simulink model "sim_dist_att_obs_paper"  (R2020a)
settings: Solver=ode4  StartTime=0.0  StopTime=30.0  FixedStep=0.01  RelTol=1e-3
values from neighbouring files (symbols this model uses):
  beta_Phi_1 = pp0 * cal_frac_squ( 3, p_p0_plus_1, q_p0_plus_1 )                          * cal_frac_squ( eps_s_bar / pi, p_p0_min_2, q_p0_min_2 )                          / ( 2 * ( 2 * pp0 - 1 ) * tanh( gamma0 * ( eps_s_bar / pi ) / 2 ) )                          - ( cal_frac_squ( 3, p_p0_plus_1, q_p0_plus_1 ) * gamma0 / ( 4 * ( 2 * pp0 -1 ) ) )                          * cal_frac_squ( eps_s_bar / pi, p_p0_min_ ...(+136 chars)    [draw_compare_dist_att_obs.m]
  beta_Phi_2 = ( 1 - pp0 ) * cal_frac_squ( 3, p_p0_plus_1, q_p0_plus_1 )                          / ( 2 * ( 1 - 2 * pp0 ) * cal_frac_squ( eps_s_bar / pi, p_p0_0, q_p0_0 ) * tanh( gamma0 * ( eps_s_bar / pi ) / 2 ) )                          - ( cal_frac_squ( 3, p_p0_plus_1, q_p0_plus_1 ) * gamma0 / ( 4 * ( 1 - 2 * pp0 ) ) )                          * cal_frac_squ( eps_s_bar / pi, p_1_min_p0, q_1_min_p0 )          ...(+112 chars)    [draw_compare_dist_att_obs.m]
  c1_diff_sigma_bar_w = diag([12; 12; 12])    [draw_compare_dist_att_obs.m]
  c1_diff_ui = diag([25; 30; 20])    [draw_compare_dist_att_obs.m]
  c2_diff_sigma_bar_w = diag([12; 12; 12])    [draw_compare_dist_att_obs.m]
  c2_diff_ui = diag([50; 50; 10])    [draw_compare_dist_att_obs.m]
  c3_diff_sigma_bar_w = diag([15; 15; 15])    [draw_compare_dist_att_obs.m]
  c3_diff_ui = diag([15; 15; 10])    [draw_compare_dist_att_obs.m]
  c_w_1 = diag( [20; 15; 15] )    [draw_compare_dist_att_obs.m]
  c_w_2 = diag( [20; 15; 15] )    [draw_compare_dist_att_obs.m]
  c_w_3 = diag( [2; 2; 2] )    [draw_compare_dist_att_obs.m]
  cS0 = diag( [4.5; 4.5; 4.5] )    [draw_compare_dist_att_obs.m]
  dw_aa_t = 0.2 * ones(3, 5) + ( 1.0 - 0.2 ) * rand(3, 5)    [draw_compare_dist_att_obs.m]
  dw_ff_t = [ 0.4 * ones(1, 5) + ( 1.0 - 0.4 ) * rand(1, 5);                      0.4 * ones(1, 5) + ( 1.0 - 0.4 ) * rand(1, 5);                      0.2 * ones(1, 5) + ( 0.6 - 0.2 ) * rand(1, 5) ]    [draw_compare_dist_att_obs.m]
  dw_phi_t = ( - pi / 2 ) * ones(3, 5) + ( pi / 2 - ( - pi / 2 ) ) * rand(3, 5)    [draw_compare_dist_att_obs.m]
  dwci_init = zeros(3,5)    [draw_compare_dist_att_obs.m]
  eps_s_bar_div_pi = eps_s_bar / pi    (= 0.03)    [draw_compare_dist_att_obs.m]
  gamma0 = 20    [draw_compare_dist_att_obs.m]
  h1w = diag([20.0; 20.0; 20.0])    [draw_compare_dist_att_obs.m]
  h2w = diag([30.0; 35.0; 35.0])    [draw_compare_dist_att_obs.m]
  h3w = diag([30.0; 25.0; 30.0])    [draw_compare_dist_att_obs.m]
  Ji = zeros(3,3,NF)    [draw_compare_dist_att_obs.m]
  k_J_0 = diag( [1; 1; 1] )    [draw_compare_dist_att_obs.m]
  Lamd_diff_sigma_bar_w = 0.8    [draw_compare_dist_att_obs.m]
  Lamd_diff_ui = 0.8    [draw_compare_dist_att_obs.m]
  mu_c_theta = 100    [draw_compare_dist_att_obs.m]
  mu_d_w = 100    [draw_compare_dist_att_obs.m]
  pos0 = zeros(3, 1)    [draw_compare_dist_att_obs.m]
  pp0 = 8 / 11    (= 0.727272727273)    [draw_compare_dist_att_obs.m]
  PZ0 = P0(3)    [draw_compare_dist_att_obs.m]
  PZ1 = 10    [draw_compare_dist_att_obs.m]
  Qci_init = repmat([1;0;0;0],1,NF)    [draw_compare_dist_att_obs.m]
  R0 = 4    [draw_compare_dist_att_obs.m]
  R1 = 8    [draw_compare_dist_att_obs.m]
  Rci_init = zeros(3,3,NF)    [draw_compare_dist_att_obs.m]
  Ri_init = zeros(3,3,NF)    [draw_compare_dist_att_obs.m]
  Rx2 = 10    [draw_compare_dist_att_obs.m]
  Ry2 = 6    [draw_compare_dist_att_obs.m]
  Rz2 = 4    [draw_compare_dist_att_obs.m]
  T0 = 0    [draw_compare_dist_att_obs.m]
  T1 = tseq1    (= 10)    [draw_compare_dist_att_obs.m]
  T2 = tseq1 + tseq12 + tseq2    (= 30)    [draw_compare_dist_att_obs.m]
  thr_p_plus_1 = cal_frac_squ( 3, p_p0_plus_1, q_p0_plus_1 )    [draw_compare_dist_att_obs.m]
  ui_init = zeros(3,NF)    [draw_compare_dist_att_obs.m]
  vel0 = zeros(3, 1)    [draw_compare_dist_att_obs.m]
  wci_init = zeros(3,5)    [draw_compare_dist_att_obs.m]
  zeta_diff_sigma_bar_w = 0.3    [draw_compare_dist_att_obs.m]
  zeta_diff_ui = 0.05    [draw_compare_dist_att_obs.m]
undefined symbols (not defined in the file or in its folder): cal_frac_squ, p_2_p0, p_alfaw1, p_alfaw2, p_beta_w_1, p_beta_w_2, p_p0_min_1, p_p0_plus_1, q_2_p0, q_alfaw1, q_alfaw2, q_beta_w_1, q_beta_w_2, q_p0_min_1, q_p0_plus_1, Qei_init, Qi_init, Rei_init, V_Phi_Rei_init, wei_init, wi_init
(part 1 of 5)
settings Model: Creator=zzy  LastModifiedBy=Hershey.A
settings DataIOCC: ReturnWorkspaceOutputs=off
settings DebuggingCC: ArithmeticOperatorsInVariantConditions=warning
settings SFSimCC: SimUseLocalCustomCode=off  CustomCodeUndefinedFunction=UseInterfaceOnly
settings RTWCC: RTWUseLocalCustomCode=off

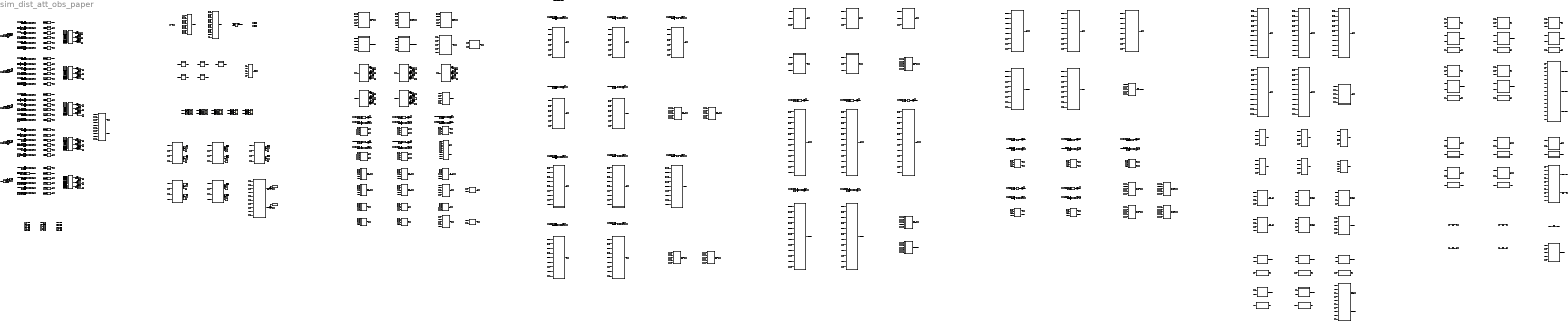
== system sim_dist_att_obs_paper ==
  Abs{,1..29} (30 alike) : Abs
  Add{10..12,14,16..18,20..22,24..26,28..29} (15 alike) : Sum
  Add{13,15,19,23,27} (5 alike) : Sum  Inputs=+-
  Clock : Clock
  Constant : Constant  Value=T1
  Constant129 : Constant  Value=R0
  Constant130 : Constant  Value=R1
  Constant131 : Constant  Value=T0
  Constant132 : Constant  Value=Rz2
  Constant133 : Constant  Value=Ry2
  Constant134 : Constant  Value=Rx2
  Constant{298,331,362,619,639} (5 alike) : Constant  Value=0
  Constant{299,411,488,556,621} (5 alike) : Constant  Value=p_p0_plus_1
  Constant{300,355,433,510,521} (5 alike) : Constant  Value=p_2_p0
  Constant{301,306,308,310,316,321,324,326,343,347,352,354,357,363,590,593,598,601,603,620,624,629,631,634,640} (25 alike) : Constant
  Constant{302,309,312..313,317,325,327..328,345..346,348,356,358..359,364..365,591..592,594,602,615..616,622..623,625,633,635..636,641..642} (30 alike) : Constant  Value=3
  Constant{303,314,318,329,349,360,595,617,626,637} (10 alike) : Constant  Value=2
  Constant{304,319,350,596,627} (5 alike) : Constant  Value=c1_diff_ui
  Constant{305,320,351,597,628} (5 alike) : Constant  Value=c2_diff_ui
  Constant{307,323,353,600,630} (5 alike) : Constant  Value=c3_diff_ui
  Constant{311,366,444,522,577} (5 alike) : Constant  Value=q_2_p0
  Constant{315,330,361,618,638} (5 alike) : Constant  Value=Lamd_diff_ui
  Constant{322,377,455,483,485,487,490,492,533,588,609,611..614} (15 alike) : Constant  Value=cS0
  Constant{332,335,337,339,341} (5 alike) : Constant  Value=p_p0_min_1
  Constant{333,388,393,461,466,468,474,481,544..545,578,583,589,599,607} (15 alike) : Constant  Value=gamma0
  Constant{334,336,338,340,342} (5 alike) : Constant  Value=q_p0_min_1
  Constant{344,392,398..399,467,473,477,480,547,555,575,581,586,605,610} (15 alike) : Constant  Value=thr_p_plus_1
  Constant{367..376,378..382} (15 alike) : Constant  Value=zeta_diff_ui
  Constant{383..387,401,413,437,447,450..452,454,457,459,484,486,489,491,493,526,530,535,539,543} (25 alike) : Constant  Value=Ji
  Constant{389,395,463,470,476} (5 alike) : Constant  Value=pp0
  Constant{390,396,464,471,478,571,579,584,604,608} (10 alike) : Constant  Value=beta_Phi_1
  Constant{391,397,465,472,479,548..549,574,580,585} (10 alike) : Constant  Value=beta_Phi_2
  Constant{394,462,469,475,482,546,576,582,587,606} (10 alike) : Constant  Value=eps_s_bar_div_pi
  Constant{400,425,445..446,448..449,453,456,458,460} (10 alike) : Constant  Value=h3w
  Constant{402,404,409,417,423} (5 alike) : Constant  Value=p_alfaw1
  Constant{403,405,412,418,424} (5 alike) : Constant  Value=mu_d_w
  Constant{406,414,419,426,429} (5 alike) : Constant  Value=q_alfaw1
  Constant{407,415,420,427,430} (5 alike) : Constant  Value=p_alfaw2
  Constant{408,416,421,428,431} (5 alike) : Constant  Value=q_alfaw2
  Constant{410,422,499,560,632} (5 alike) : Constant  Value=q_p0_plus_1
  Constant{432,435,438,440,442} (5 alike) : Constant  Value=h1w
  Constant{434,436,439,441,443} (5 alike) : Constant  Value=h2w
  Constant{494,500,505,511,516} (5 alike) : Constant  Value=p_beta_w_1
  Constant{495,501,506,512,517} (5 alike) : Constant  Value=q_beta_w_1
  Constant{496,502,507,513,518} (5 alike) : Constant  Value=p_beta_w_2
  Constant{497,503,508,514,519} (5 alike) : Constant  Value=q_beta_w_2
  Constant{498,504,509,515,520} (5 alike) : Constant  Value=mu_c_theta
  Constant{523,527,531,536,540} (5 alike) : Constant  Value=c_w_1
  Constant{524,528,532,537,541} (5 alike) : Constant  Value=c_w_2
  Constant{525,529,534,538,542} (5 alike) : Constant  Value=c_w_3
  Constant{550..554} (5 alike) : Constant  Value=k_J_0
  Constant{557,561,564,567,570} (5 alike) : Constant  Value=dw_aa_t
  Constant{558,562,565,568,572} (5 alike) : Constant  Value=dw_ff_t
  Constant{559,563,566,569,573} (5 alike) : Constant  Value=dw_phi_t
  Constant64 : Constant  Value=T2
  Constant65 : Constant  Value=R0
  Constant66 : Constant  Value=R1
  Constant67 : Constant  Value=Rx2
  Constant68 : Constant  Value=Ry2
  Constant69 : Constant  Value=Rz2
  Constant70 : Constant  Value=T2
  Constant71 : Constant  Value=T1
  Constant72 : Constant  Value=PZ0
  Constant73 : Constant  Value=PZ1
  Demux{,1,22,98..141} (47 alike) : Demux  Outputs=3
  Display{96..172} (77 alike) : Display
  Integrator{1..15,46..50} (20 alike) : Integrator  InitialCondition=zeros(3,1)
  Integrator17 : Integrator  InitialCondition=V_Phi_Rei_init(:,2)
  Integrator19 : Integrator  InitialCondition=V_Phi_Rei_init(:,3)
  Integrator20 : Integrator  InitialCondition=V_Phi_Rei_init(:,1)
  Integrator21 : Integrator  InitialCondition=wi_init(:,1)
  Integrator22 : Integrator  InitialCondition=wi_init(:,2)
  Integrator23 : Integrator  InitialCondition=wi_init(:,3)
  Integrator24 : Integrator  InitialCondition=wi_init(:,4)
  Integrator25 : Integrator  InitialCondition=wi_init(:,5)
  Integrator26 : Integrator  InitialCondition=Qi_init(:,1)
  Integrator27 : Integrator  InitialCondition=Qi_init(:,2)
  Integrator28 : Integrator  InitialCondition=Qi_init(:,3)
  Integrator29 : Integrator  InitialCondition=Qi_init(:,4)
  Integrator30 : Integrator  InitialCondition=Qi_init(:,5)
  Integrator31 : Integrator  InitialCondition=Qei_init(:,1)
  Integrator32 : Integrator  InitialCondition=Qei_init(:,2)
  Integrator33 : Integrator  InitialCondition=Qei_init(:,3)
  Integrator34 : Integrator  InitialCondition=Qei_init(:,4)
  Integrator35 : Integrator  InitialCondition=Qei_init(:,5)
  Integrator42 : Integrator  InitialCondition=V_Phi_Rei_init(:,4)
  Integrator44 : Integrator  InitialCondition=V_Phi_Rei_init(:,5)
  Interpreted MATLAB Function{,61..124} (65 alike) : MATLABFcn  MATLABFcn=cal_frac_squ(u(1:3),u(4),u(5))
  Memory : Memory  InitialCondition=ui_init
  Memory{9..11,13,18..25} (12 alike) : Memory  InitialCondition=zeros(3,5)
  Memory12 : Memory  InitialCondition=V_Phi_Rei_init
  Memory14 : Memory  InitialCondition=wci_init
  Memory15 : Memory  InitialCondition=dwci_init
  Memory16 : Memory  InitialCondition=Qci_init
  Memory17 : Memory  InitialCondition=Rci_init
  Memory3 : Memory  InitialCondition=Qi_init
  Memory4 : Memory  InitialCondition=Ri_init
  Memory5 : Memory  InitialCondition=wi_init
  Memory6 : Memory  InitialCondition=wei_init
  Memory7 : Memory  InitialCondition=Qei_init
  Memory8 : Memory  InitialCondition=Rei_init
  Mux{136..170,180,187..215} (65 alike) : Mux  Inputs=3
  Mux{171..179,181..186} (15 alike) : Mux  Inputs=2
  Product{,1..9} (10 alike) : Product
  Qei dynam agent 1 : MATLAB Function  TreatAsAtomicUnit=on
  Qei dynam agent 2 : MATLAB Function  TreatAsAtomicUnit=on
  Qei dynam agent 3 : MATLAB Function  TreatAsAtomicUnit=on
  Qei dynam agent 4 : MATLAB Function  TreatAsAtomicUnit=on
  Qei dynam agent 5 : MATLAB Function  TreatAsAtomicUnit=on
  Qi dynam agent 1 : MATLAB Function  TreatAsAtomicUnit=on
  Qi dynam agent 2 : MATLAB Function  TreatAsAtomicUnit=on
  Qi dynam agent 3 : MATLAB Function  TreatAsAtomicUnit=on
  Qi dynam agent 4 : MATLAB Function  TreatAsAtomicUnit=on
  Qi dynam agent 5 : MATLAB Function  TreatAsAtomicUnit=on
  Scope{1..2,13..15} (5 alike) : Scope  NumInputPorts=3
  Step : Step  Time=T1+0.01  SampleTime=0
  To Workspace23 : ToWorkspace  VariableName=wci  SampleTime=-1
  To Workspace24 : ToWorkspace  VariableName=V_Phi_Rei  SampleTime=-1
  To Workspace25 : ToWorkspace  VariableName=dwi_tilt  SampleTime=-1
  To Workspace26 : ToWorkspace  VariableName=Qci  SampleTime=-1
  To Workspace27 : ToWorkspace  VariableName=sigma_bar_w_hat  SampleTime=-1
  To Workspace28 : ToWorkspace  VariableName=wei  SampleTime=-1
  To Workspace29 : ToWorkspace  VariableName=sigma_w  SampleTime=-1
  To Workspace30 : ToWorkspace  VariableName=sigma_bar_w  SampleTime=-1
  To Workspace31 : ToWorkspace  VariableName=Phi_psi_e  SampleTime=-1
  To Workspace32 : ToWorkspace  VariableName=Phi_bar_psi_e  SampleTime=-1
  To Workspace33 : ToWorkspace  VariableName=Qei  SampleTime=-1
  To Workspace34 : ToWorkspace  VariableName=wi  SampleTime=-1
  To Workspace35 : ToWorkspace  VariableName=Qi  SampleTime=-1
  To Workspace36 : ToWorkspace  VariableName=S_bar  SampleTime=-1
  To Workspace37 : ToWorkspace  VariableName=Si  SampleTime=-1
  To Workspace38 : ToWorkspace  VariableName=dwi  SampleTime=-1
  To Workspace39 : ToWorkspace  VariableName=dwi_hat  SampleTime=-1
  cal Fi_S agent 1 : MATLAB Function  TreatAsAtomicUnit=on
  cal Fi_S agent 2 : MATLAB Function  TreatAsAtomicUnit=on
  cal Fi_S agent 3 : MATLAB Function  TreatAsAtomicUnit=on
  cal Fi_S agent 4 : MATLAB Function  TreatAsAtomicUnit=on
  cal Fi_S agent 5 : MATLAB Function  TreatAsAtomicUnit=on
  cal Phi_bar_psi_e agent 1 : MATLAB Function  TreatAsAtomicUnit=on
  cal Phi_bar_psi_e agent 2 : MATLAB Function  TreatAsAtomicUnit=on
  cal Phi_bar_psi_e agent 3 : MATLAB Function  TreatAsAtomicUnit=on
  cal Phi_bar_psi_e agent 4 : MATLAB Function  TreatAsAtomicUnit=on
  cal Phi_bar_psi_e agent 5 : MATLAB Function  TreatAsAtomicUnit=on
  cal Phi_psi_e agent 1 : MATLAB Function  TreatAsAtomicUnit=on
  cal Phi_psi_e agent 2 : MATLAB Function  TreatAsAtomicUnit=on
  cal Phi_psi_e agent 3 : MATLAB Function  TreatAsAtomicUnit=on
  cal Phi_psi_e agent 4 : MATLAB Function  TreatAsAtomicUnit=on
  cal Phi_psi_e agent 5 : MATLAB Function  TreatAsAtomicUnit=on
  cal Qci agent 1 : MATLAB Function  TreatAsAtomicUnit=on
  cal Qci agent 2 : MATLAB Function  TreatAsAtomicUnit=on
  cal Qci agent 3 : MATLAB Function  TreatAsAtomicUnit=on
  cal Qci agent 4 : MATLAB Function  TreatAsAtomicUnit=on
  cal Qci agent 5 : MATLAB Function  TreatAsAtomicUnit=on
  cal Rci agent 1 : MATLAB Function  TreatAsAtomicUnit=on
  cal Rci agent 2 : MATLAB Function  TreatAsAtomicUnit=on
  cal Rci agent 3 : MATLAB Function  TreatAsAtomicUnit=on
  cal Rci agent 4 : MATLAB Function  TreatAsAtomicUnit=on
  cal Rci agent 5 : MATLAB Function  TreatAsAtomicUnit=on
  cal Rei agent 1 : MATLAB Function  TreatAsAtomicUnit=on
  cal Rei agent 2 : MATLAB Function  TreatAsAtomicUnit=on
  cal Rei agent 3 : MATLAB Function  TreatAsAtomicUnit=on
  cal Rei agent 4 : MATLAB Function  TreatAsAtomicUnit=on
  cal Rei agent 5 : MATLAB Function  TreatAsAtomicUnit=on
  cal Ri agent 1 : MATLAB Function  TreatAsAtomicUnit=on
  cal Ri agent 2 : MATLAB Function  TreatAsAtomicUnit=on
  cal Ri agent 3 : MATLAB Function  TreatAsAtomicUnit=on
  cal Ri agent 4 : MATLAB Function  TreatAsAtomicUnit=on
  cal Ri agent 5 : MATLAB Function  TreatAsAtomicUnit=on
  cal S_bar agent 1 : MATLAB Function  TreatAsAtomicUnit=on
  cal S_bar agent 2 : MATLAB Function  TreatAsAtomicUnit=on
  cal S_bar agent 3 : MATLAB Function  TreatAsAtomicUnit=on
  cal S_bar agent 4 : MATLAB Function  TreatAsAtomicUnit=on
  cal S_bar agent 5 : MATLAB Function  TreatAsAtomicUnit=on
  cal Si agent 1 : MATLAB Function  TreatAsAtomicUnit=on
  cal Si agent 2 : MATLAB Function  TreatAsAtomicUnit=on
  cal Si agent 3 : MATLAB Function  TreatAsAtomicUnit=on
  cal Si agent 4 : MATLAB Function  TreatAsAtomicUnit=on
  cal Si agent 5 : MATLAB Function  TreatAsAtomicUnit=on
  cal abs 61 : MATLAB Function  TreatAsAtomicUnit=on
  cal abs 62 : MATLAB Function  TreatAsAtomicUnit=on
  cal abs 63 : MATLAB Function  TreatAsAtomicUnit=on
  cal abs 64 : MATLAB Function  TreatAsAtomicUnit=on
  cal abs 65 : MATLAB Function  TreatAsAtomicUnit=on
  cal abs 66 : MATLAB Function  TreatAsAtomicUnit=on
  cal abs 67 : MATLAB Function  TreatAsAtomicUnit=on
  cal abs 68 : MATLAB Function  TreatAsAtomicUnit=on
  cal abs 69 : MATLAB Function  TreatAsAtomicUnit=on
  cal abs 70 : MATLAB Function  TreatAsAtomicUnit=on
  cal abs 71 : MATLAB Function  TreatAsAtomicUnit=on
  cal abs 72 : MATLAB Function  TreatAsAtomicUnit=on
  cal abs 73 : MATLAB Function  TreatAsAtomicUnit=on
  cal abs 74 : MATLAB Function  TreatAsAtomicUnit=on
  cal abs 75 : MATLAB Function  TreatAsAtomicUnit=on
  cal abs 76 : MATLAB Function  TreatAsAtomicUnit=on
  cal abs 77 : MATLAB Function  TreatAsAtomicUnit=on
  cal abs 78 : MATLAB Function  TreatAsAtomicUnit=on
  cal abs 79 : MATLAB Function  TreatAsAtomicUnit=on
  cal abs 80 : MATLAB Function  TreatAsAtomicUnit=on
  cal abs 81 : MATLAB Function  TreatAsAtomicUnit=on
  cal abs 82 : MATLAB Function  TreatAsAtomicUnit=on
  cal abs 83 : MATLAB Function  TreatAsAtomicUnit=on
  cal abs 84 : MATLAB Function  TreatAsAtomicUnit=on
  cal abs 85 : MATLAB Function  TreatAsAtomicUnit=on
  cal abs 86 : MATLAB Function  TreatAsAtomicUnit=on
  cal abs 87 : MATLAB Function  TreatAsAtomicUnit=on
  cal abs 88 : MATLAB Function  TreatAsAtomicUnit=on
  cal abs 89 : MATLAB Function  TreatAsAtomicUnit=on
  cal abs 90 : MATLAB Function  TreatAsAtomicUnit=on
  cal abs 91 : MATLAB Function  TreatAsAtomicUnit=on
  cal abs 92 : MATLAB Function  TreatAsAtomicUnit=on
  cal abs 93 : MATLAB Function  TreatAsAtomicUnit=on
  cal abs 94 : MATLAB Function  TreatAsAtomicUnit=on
  cal abs 95 : MATLAB Function  TreatAsAtomicUnit=on
  cal combine sigma_bar_w_tilt : MATLAB Function  TreatAsAtomicUnit=on
  cal d_sigma_w agent 1 : MATLAB Function  TreatAsAtomicUnit=on
  cal d_sigma_w agent 2 : MATLAB Function  TreatAsAtomicUnit=on
  cal d_sigma_w agent 3 : MATLAB Function  TreatAsAtomicUnit=on
  cal d_sigma_w agent 4 : MATLAB Function  TreatAsAtomicUnit=on
  cal d_sigma_w agent 5 : MATLAB Function  TreatAsAtomicUnit=on
  cal d_theta_hat : MATLAB Function  TreatAsAtomicUnit=on
  cal d_theta_hat1 : MATLAB Function  TreatAsAtomicUnit=on
  cal d_theta_hat2 : MATLAB Function  TreatAsAtomicUnit=on
  cal d_theta_hat3 : MATLAB Function  TreatAsAtomicUnit=on
  cal d_theta_hat4 : MATLAB Function  TreatAsAtomicUnit=on
  cal differentiator d_sigma_bar_w_hat agent 1 : Subsystem
  cal differentiator d_sigma_bar_w_hat agent 2 : Subsystem
  cal differentiator d_sigma_bar_w_hat agent 3 : Subsystem
  cal differentiator d_sigma_bar_w_hat agent 4 : Subsystem
  cal differentiator d_sigma_bar_w_hat agent 5 : Subsystem
  cal divide pi : MATLAB Function  TreatAsAtomicUnit=on
  cal dw_hat agent 1 : MATLAB Function  TreatAsAtomicUnit=on
  cal dw_hat agent 2 : MATLAB Function  TreatAsAtomicUnit=on
  cal dw_hat agent 3 : MATLAB Function  TreatAsAtomicUnit=on
  cal dw_hat agent 4 : MATLAB Function  TreatAsAtomicUnit=on
  cal dw_hat agent 5 : MATLAB Function  TreatAsAtomicUnit=on
  cal error dw_tilt : MATLAB Function  TreatAsAtomicUnit=on
  cal sig : MATLAB Function  TreatAsAtomicUnit=on
  cal sig1 : MATLAB Function  TreatAsAtomicUnit=on
  cal sig10 : MATLAB Function  TreatAsAtomicUnit=on
  cal sig11 : MATLAB Function  TreatAsAtomicUnit=on
  cal sig12 : MATLAB Function  TreatAsAtomicUnit=on
  cal sig13 : MATLAB Function  TreatAsAtomicUnit=on
  cal sig14 : MATLAB Function  TreatAsAtomicUnit=on
  cal sig15 : MATLAB Function  TreatAsAtomicUnit=on
  cal sig16 : MATLAB Function  TreatAsAtomicUnit=on
  cal sig17 : MATLAB Function  TreatAsAtomicUnit=on
  cal sig18 : MATLAB Function  TreatAsAtomicUnit=on
  cal sig19 : MATLAB Function  TreatAsAtomicUnit=on
  cal sig2 : MATLAB Function  TreatAsAtomicUnit=on
  cal sig20 : MATLAB Function  TreatAsAtomicUnit=on
  cal sig21 : MATLAB Function  TreatAsAtomicUnit=on
  cal sig22 : MATLAB Function  TreatAsAtomicUnit=on
  cal sig23 : MATLAB Function  TreatAsAtomicUnit=on
  cal sig24 : MATLAB Function  TreatAsAtomicUnit=on
  cal sig25 : MATLAB Function  TreatAsAtomicUnit=on
  cal sig26 : MATLAB Function  TreatAsAtomicUnit=on
  cal sig27 : MATLAB Function  TreatAsAtomicUnit=on
  cal sig28 : MATLAB Function  TreatAsAtomicUnit=on
  cal sig29 : MATLAB Function  TreatAsAtomicUnit=on
  cal sig3 : MATLAB Function  TreatAsAtomicUnit=on
  cal sig4 : MATLAB Function  TreatAsAtomicUnit=on
  cal sig5 : MATLAB Function  TreatAsAtomicUnit=on
  cal sig6 : MATLAB Function  TreatAsAtomicUnit=on
  cal sig7 : MATLAB Function  TreatAsAtomicUnit=on
  cal sig8 : MATLAB Function  TreatAsAtomicUnit=on
  cal sig9 : MATLAB Function  TreatAsAtomicUnit=on
  cal sigma_bar_w_hat agent 1 : MATLAB Function  TreatAsAtomicUnit=on
  cal sigma_bar_w_hat agent 2 : MATLAB Function  TreatAsAtomicUnit=on
  cal sigma_bar_w_hat agent 3 : MATLAB Function  TreatAsAtomicUnit=on
  cal sigma_bar_w_hat agent 4 : MATLAB Function  TreatAsAtomicUnit=on
  cal sigma_bar_w_hat agent 5 : MATLAB Function  TreatAsAtomicUnit=on
  cal sigma_w_bar : MATLAB Function  TreatAsAtomicUnit=on
  cal taui agent 1 : MATLAB Function  TreatAsAtomicUnit=on
  cal taui agent 2 : MATLAB Function  TreatAsAtomicUnit=on
  cal taui agent 3 : MATLAB Function  TreatAsAtomicUnit=on
  cal taui agent 4 : MATLAB Function  TreatAsAtomicUnit=on
  cal taui agent 5 : MATLAB Function  TreatAsAtomicUnit=on
  cal theta_Si_beta_w agent 1 : MATLAB Function  TreatAsAtomicUnit=on
  cal theta_Si_beta_w agent 2 : MATLAB Function  TreatAsAtomicUnit=on
  cal theta_Si_beta_w agent 3 : MATLAB Function  TreatAsAtomicUnit=on
  cal theta_Si_beta_w agent 4 : MATLAB Function  TreatAsAtomicUnit=on
  cal theta_Si_beta_w agent 5 : MATLAB Function  TreatAsAtomicUnit=on
  cal theta_sigma_bar_w_tilt agent 1 : MATLAB Function  TreatAsAtomicUnit=on
  cal theta_sigma_bar_w_tilt agent 2 : MATLAB Function  TreatAsAtomicUnit=on
  cal theta_sigma_bar_w_tilt agent 3 : MATLAB Function  TreatAsAtomicUnit=on
  cal theta_sigma_bar_w_tilt agent 4 : MATLAB Function  TreatAsAtomicUnit=on
  cal theta_sigma_bar_w_tilt agent 5 : MATLAB Function  TreatAsAtomicUnit=on
  cal wci dwci agent 1 : MATLAB Function  TreatAsAtomicUnit=on
  cal wci dwci agent 2 : MATLAB Function  TreatAsAtomicUnit=on
  cal wci dwci agent 3 : MATLAB Function  TreatAsAtomicUnit=on
  cal wci dwci agent 4 : MATLAB Function  TreatAsAtomicUnit=on
  cal wci dwci agent 5 : MATLAB Function  TreatAsAtomicUnit=on
  cal wei agent 1 : MATLAB Function  TreatAsAtomicUnit=on
  cal wei agent 2 : MATLAB Function  TreatAsAtomicUnit=on
  cal wei agent 3 : MATLAB Function  TreatAsAtomicUnit=on
  cal wei agent 4 : MATLAB Function  TreatAsAtomicUnit=on
  cal wei agent 5 : MATLAB Function  TreatAsAtomicUnit=on
  choose ksi_est_err 41 : MATLAB Function  TreatAsAtomicUnit=on
  choose ksi_est_err 42 : MATLAB Function  TreatAsAtomicUnit=on
  choose ksi_est_err 43 : MATLAB Function  TreatAsAtomicUnit=on
  choose ksi_est_err 44 : MATLAB Function  TreatAsAtomicUnit=on
  choose ksi_est_err 45 : MATLAB Function  TreatAsAtomicUnit=on
  choose ksi_est_err 46 : MATLAB Function  TreatAsAtomicUnit=on
  choose ksi_est_err 47 : MATLAB Function  TreatAsAtomicUnit=on
  choose ksi_est_err 48 : MATLAB Function  TreatAsAtomicUnit=on
  choose ksi_est_err 49 : MATLAB Function  TreatAsAtomicUnit=on
  choose ksi_est_err 50 : MATLAB Function  TreatAsAtomicUnit=on
  choose ksi_est_err 51 : MATLAB Function  TreatAsAtomicUnit=on
  choose ksi_est_err 52 : MATLAB Function  TreatAsAtomicUnit=on
  choose ksi_est_err 53 : MATLAB Function  TreatAsAtomicUnit=on
  choose ksi_est_err 54 : MATLAB Function  TreatAsAtomicUnit=on
  choose ksi_est_err 55 : MATLAB Function  TreatAsAtomicUnit=on
  choose ksi_est_err 56 : MATLAB Function  TreatAsAtomicUnit=on
  choose ksi_est_err 57 : MATLAB Function  TreatAsAtomicUnit=on
  choose ksi_est_err 58 : MATLAB Function  TreatAsAtomicUnit=on
  choose ksi_est_err 59 : MATLAB Function  TreatAsAtomicUnit=on
  choose ksi_est_err 60 : MATLAB Function  TreatAsAtomicUnit=on
  choose ksi_est_err 61 : MATLAB Function  TreatAsAtomicUnit=on
  choose ksi_est_err 62 : MATLAB Function  TreatAsAtomicUnit=on
  choose ksi_est_err 63 : MATLAB Function  TreatAsAtomicUnit=on
  choose ksi_est_err 64 : MATLAB Function  TreatAsAtomicUnit=on
  choose ksi_est_err 65 : MATLAB Function  TreatAsAtomicUnit=on
  choose ksi_est_err 66 : MATLAB Function  TreatAsAtomicUnit=on
  choose ksi_est_err 67 : MATLAB Function  TreatAsAtomicUnit=on
  choose ksi_est_err 68 : MATLAB Function  TreatAsAtomicUnit=on
  choose ksi_est_err 69 : MATLAB Function  TreatAsAtomicUnit=on
  choose ksi_est_err 70 : MATLAB Function  TreatAsAtomicUnit=on
  choose ksi_est_err 71 : MATLAB Function  TreatAsAtomicUnit=on
  choose ksi_est_err 72 : MATLAB Function  TreatAsAtomicUnit=on
  choose ksi_est_err 73 : MATLAB Function  TreatAsAtomicUnit=on
  choose ksi_est_err 74 : MATLAB Function  TreatAsAtomicUnit=on
  choose ksi_est_err 75 : MATLAB Function  TreatAsAtomicUnit=on
  choose ui agent 1 : MATLAB Function  TreatAsAtomicUnit=on
  choose ui agent 2 : MATLAB Function  TreatAsAtomicUnit=on
  choose ui agent 3 : MATLAB Function  TreatAsAtomicUnit=on
  choose ui agent 4 : MATLAB Function  TreatAsAtomicUnit=on
  choose ui agent 5 : MATLAB Function  TreatAsAtomicUnit=on
  combine Fi_S : MATLAB Function  TreatAsAtomicUnit=on
  combine Phi_bar_psi_e : MATLAB Function  TreatAsAtomicUnit=on
  combine Phi_psi_e : MATLAB Function  TreatAsAtomicUnit=on
  combine Qci Rci : MATLAB Function  TreatAsAtomicUnit=on
  combine Qci Rci1 : MATLAB Function  TreatAsAtomicUnit=on
  combine Qi Ri : MATLAB Function  TreatAsAtomicUnit=on
  combine S_bar : MATLAB Function  TreatAsAtomicUnit=on
  combine Si : MATLAB Function  TreatAsAtomicUnit=on
  combine Si_squ_beta_w_1 : MATLAB Function  TreatAsAtomicUnit=on
  combine Si_squ_beta_w_2 : MATLAB Function  TreatAsAtomicUnit=on
  combine V_Phi_Rei_squ_2p : MATLAB Function  TreatAsAtomicUnit=on
  combine V_Phi_Rei_squ_p_min_1 : MATLAB Function  TreatAsAtomicUnit=on
  combine V_Phi_Rei_squ_p_plus_1 : MATLAB Function  TreatAsAtomicUnit=on
  combine d_sigma_bar_v_est1 : MATLAB Function  TreatAsAtomicUnit=on
  combine duihat d2uihat : MATLAB Function  TreatAsAtomicUnit=on
  combine dw_hat : MATLAB Function  TreatAsAtomicUnit=on
  combine dwi : MATLAB Function  TreatAsAtomicUnit=on
  combine norminal formation control input : MATLAB Function  TreatAsAtomicUnit=on
  combine sigma_bar_w_hat : MATLAB Function  TreatAsAtomicUnit=on
  combine sigma_w : MATLAB Function  TreatAsAtomicUnit=on
  combine tau : MATLAB Function  TreatAsAtomicUnit=on
  combine tau1 : MATLAB Function  TreatAsAtomicUnit=on
  combine theta_Si_beta_w_1 : MATLAB Function  TreatAsAtomicUnit=on
  combine theta_Si_beta_w_2 : MATLAB Function  TreatAsAtomicUnit=on
  combine theta_sigma_bar_w_tilt : MATLAB Function  TreatAsAtomicUnit=on
  combine wci dwci : MATLAB Function  TreatAsAtomicUnit=on
  combine wei Qei Rei : MATLAB Function  TreatAsAtomicUnit=on
  control input generator agent 1 : MATLAB Function  TreatAsAtomicUnit=on
  control input generator agent 2 : MATLAB Function  TreatAsAtomicUnit=on
  control input generator agent 3 : MATLAB Function  TreatAsAtomicUnit=on
  control input generator agent 4 : MATLAB Function  TreatAsAtomicUnit=on
  control input generator agent 5 : MATLAB Function  TreatAsAtomicUnit=on
  d2_sigma_bar_w_est_{1..5} (5 alike) : Scope  NumInputPorts=3
  d2_ui_hat_node_{1..5} (5 alike) : Scope  NumInputPorts=3
  d_sigma_bar_w_est_{1..5} (5 alike) : Scope  NumInputPorts=3
  d_ui_hat_node_{1..5} (5 alike) : Scope  NumInputPorts=3
  dwci_node_{1..5} (5 alike) : Scope  NumInputPorts=3
  eta_0 : Scope  NumInputPorts=3
  generate angular rate disturbance agent 1 : MATLAB Function  TreatAsAtomicUnit=on
  generate angular rate disturbance agent 2 : MATLAB Function  TreatAsAtomicUnit=on
  generate angular rate disturbance agent 3 : MATLAB Function  TreatAsAtomicUnit=on
  generate angular rate disturbance agent 4 : MATLAB Function  TreatAsAtomicUnit=on
  generate angular rate disturbance agent 5 : MATLAB Function  TreatAsAtomicUnit=on
  ksi_0 : Scope  NumInputPorts=3
  leader control input : MATLAB Function  TreatAsAtomicUnit=on
  leader eta0 Integrator : Integrator  ExternalReset=rising  InitialConditionSource=external  InitialCondition=vel0
  leader ksi0 Integrator : Integrator  InitialCondition=pos0
  process velocity : MATLAB Function  TreatAsAtomicUnit=on
  sigma_bar_w_hat Integrator {1..5} (5 alike) : Integrator  InitialCondition=zeros(3,1)
  trans to column100 : MATLAB Function  TreatAsAtomicUnit=on
  trans to column101 : MATLAB Function  TreatAsAtomicUnit=on
  trans to column102 : MATLAB Function  TreatAsAtomicUnit=on
  trans to column103 : MATLAB Function  TreatAsAtomicUnit=on
  trans to column104 : MATLAB Function  TreatAsAtomicUnit=on
  trans to column105 : MATLAB Function  TreatAsAtomicUnit=on
  trans to column106 : MATLAB Function  TreatAsAtomicUnit=on
  trans to column107 : MATLAB Function  TreatAsAtomicUnit=on
  trans to column108 : MATLAB Function  TreatAsAtomicUnit=on
  trans to column109 : MATLAB Function  TreatAsAtomicUnit=on
  trans to column110 : MATLAB Function  TreatAsAtomicUnit=on
  trans to column111 : MATLAB Function  TreatAsAtomicUnit=on
  trans to column112 : MATLAB Function  TreatAsAtomicUnit=on
  trans to column113 : MATLAB Function  TreatAsAtomicUnit=on
  trans to column114 : MATLAB Function  TreatAsAtomicUnit=on
  trans to column115 : MATLAB Function  TreatAsAtomicUnit=on
  trans to column116 : MATLAB Function  TreatAsAtomicUnit=on
  trans to column117 : MATLAB Function  TreatAsAtomicUnit=on
  trans to column118 : MATLAB Function  TreatAsAtomicUnit=on
  trans to column119 : MATLAB Function  TreatAsAtomicUnit=on
  trans to column120 : MATLAB Function  TreatAsAtomicUnit=on
  trans to column121 : MATLAB Function  TreatAsAtomicUnit=on
  trans to column122 : MATLAB Function  TreatAsAtomicUnit=on
  trans to column123 : MATLAB Function  TreatAsAtomicUnit=on
  trans to column124 : MATLAB Function  TreatAsAtomicUnit=on
  trans to column125 : MATLAB Function  TreatAsAtomicUnit=on
  trans to column61 : MATLAB Function  TreatAsAtomicUnit=on
  trans to column62 : MATLAB Function  TreatAsAtomicUnit=on
  trans to column63 : MATLAB Function  TreatAsAtomicUnit=on
  trans to column64 : MATLAB Function  TreatAsAtomicUnit=on
  trans to column65 : MATLAB Function  TreatAsAtomicUnit=on
  trans to column66 : MATLAB Function  TreatAsAtomicUnit=on
  trans to column67 : MATLAB Function  TreatAsAtomicUnit=on
  trans to column68 : MATLAB Function  TreatAsAtomicUnit=on
  trans to column69 : MATLAB Function  TreatAsAtomicUnit=on
  trans to column70 : MATLAB Function  TreatAsAtomicUnit=on
  trans to column71 : MATLAB Function  TreatAsAtomicUnit=on
  trans to column72 : MATLAB Function  TreatAsAtomicUnit=on
  trans to column73 : MATLAB Function  TreatAsAtomicUnit=on
  trans to column74 : MATLAB Function  TreatAsAtomicUnit=on
  trans to column75 : MATLAB Function  TreatAsAtomicUnit=on
  trans to column76 : MATLAB Function  TreatAsAtomicUnit=on
  trans to column77 : MATLAB Function  TreatAsAtomicUnit=on
  trans to column78 : MATLAB Function  TreatAsAtomicUnit=on
  trans to column79 : MATLAB Function  TreatAsAtomicUnit=on
  trans to column80 : MATLAB Function  TreatAsAtomicUnit=on
  trans to column81 : MATLAB Function  TreatAsAtomicUnit=on
  trans to column82 : MATLAB Function  TreatAsAtomicUnit=on
  trans to column83 : MATLAB Function  TreatAsAtomicUnit=on
  trans to column84 : MATLAB Function  TreatAsAtomicUnit=on
  trans to column85 : MATLAB Function  TreatAsAtomicUnit=on
  trans to column86 : MATLAB Function  TreatAsAtomicUnit=on
  trans to column87 : MATLAB Function  TreatAsAtomicUnit=on
  trans to column88 : MATLAB Function  TreatAsAtomicUnit=on
  trans to column89 : MATLAB Function  TreatAsAtomicUnit=on
  trans to column90 : MATLAB Function  TreatAsAtomicUnit=on
  trans to column91 : MATLAB Function  TreatAsAtomicUnit=on
  trans to column92 : MATLAB Function  TreatAsAtomicUnit=on
  trans to column93 : MATLAB Function  TreatAsAtomicUnit=on
  trans to column94 : MATLAB Function  TreatAsAtomicUnit=on
  trans to column95 : MATLAB Function  TreatAsAtomicUnit=on
  trans to column96 : MATLAB Function  TreatAsAtomicUnit=on
  trans to column97 : MATLAB Function  TreatAsAtomicUnit=on
  trans to column98 : MATLAB Function  TreatAsAtomicUnit=on
  trans to column99 : MATLAB Function  TreatAsAtomicUnit=on
  ui_tilt_node_{1..5} (5 alike) : Scope  NumInputPorts=3
  wci_node_{1..5} (5 alike) : Scope  NumInputPorts=3
  wi dynam agent 1 : MATLAB Function  TreatAsAtomicUnit=on
  wi dynam agent 2 : MATLAB Function  TreatAsAtomicUnit=on
  wi dynam agent 3 : MATLAB Function  TreatAsAtomicUnit=on
  wi dynam agent 4 : MATLAB Function  TreatAsAtomicUnit=on
  wi dynam agent 5 : MATLAB Function  TreatAsAtomicUnit=on
  wires:
  Constant558/1 -> generate angular rate disturbance agent 1/2(dw_ff_t)
  generate angular rate disturbance agent 5/1(dw_5) -> [dw_5]
  [tsim] -> generate angular rate disturbance agent 5/4(t)
  Memory13/1 -> [V_Phi_Rei_squ_2p_vec]
  trans to column95/1(y) -> [V_Phi_Rei_squ_2p_node_5], Display123/1
  Memory14/1 -> Display100/1, [wci_vec]
  Constant586/1 -> cal Phi_psi_e agent 4/4(thr_p_plus_1)
  [ui_tilt_node_3] -> Abs13/1
  [Phi_bar_psi_e_vec] -> cal Fi_S agent 4/8(Phi_bar_psi_e_vec)
  trans to column104/1(y) -> [Si_squ_beta_w_1_node_2], Display157/1
  [wi_vec] -> Qi dynam agent 3/2(wi_vec)
  [Fi_S_vec] -> cal taui agent 1/8(Fi_S_vec)
  Memory20/1 -> [Fi_S_vec]
  [S_bar_node_4] -> combine S_bar/4(S_bar_node_4)
  [sigma_w_5] -> combine sigma_w/5(sigma_w_5)
  Memory11/1 -> [S_bar_vec]
  [theta_Si_beta_w_1_vec] -> cal taui agent 1/9(theta_Si_beta_w_1_vec)
  cal sigma_bar_w_hat agent 3/1(d_sigma_bar_w_hat_3) -> sigma_bar_w_hat Integrator 3/1
  Interpreted MATLAB Function61/1 -> trans to column61/1(x)
  Constant436/1 -> cal sigma_bar_w_hat agent 2/2(h2w)
  [dwci_vec] -> cal Fi_S agent 3/6(dwci_vec)
  Demux/2 -> Mux172/1
  Constant351/1 -> cal d_theta_hat4/2(c2)
  [V_Phi_Rei_squ_2p_vec] -> cal Phi_psi_e agent 4/9(V_Phi_Rei_squ_2p_vec)
  Constant588/1 -> cal S_bar agent 1/1(cS0)
  trans to column118/1(y) -> [Si_squ_beta_w_1_node_3], Display159/1
  [V_Phi_Rei_div_pi_vec] -> choose ksi_est_err 55/1(x)
  [V_Phi_Rei_squ_2p_vec] -> cal Phi_psi_e agent 3/9(V_Phi_Rei_squ_2p_vec)
  Constant604/1 -> cal Phi_psi_e agent 4/1(beta_Phi_1)
  [S_bar_vec] -> cal Phi_psi_e agent 4/6(S_bar_vec)
  Constant547/1 -> cal Phi_psi_e agent 3/4(thr_p_plus_1)
  combine Phi_psi_e/1(Phi_psi_e_vec) -> Memory18/1
  Constant454/1 -> cal dw_hat agent 4/2(Ji)
  [d2_ui_hat_node_4] -> cal d_theta_hat3/12(d2ui_hat)
  Constant520/1 -> cal theta_Si_beta_w agent 5/1(mu_c_theta)
  [ui_squ_1_node_3] -> cal sig14/1(x)
  cal d_sigma_w agent 4/1(d_sigma_w_4) -> Integrator49/1
  choose ksi_est_err 43/1(y) -> cal abs 63/1(x)
  Constant584/1 -> cal Phi_psi_e agent 3/1(beta_Phi_1)
  cal Si agent 4/1(Si_4) -> [Si_4]
  Constant546/1 -> cal Phi_psi_e agent 2/5(eps_s_bar_div_pi)
  [Si_1] -> combine Si/1(Si_1)
  [V_Phi_Rei_div_pi_vec] -> cal Phi_psi_e agent 2/7(V_Phi_Rei_div_pi_vec)
  [dw_vec] -> wi dynam agent 5/4(dw_vec)
  [Phi_bar_psi_e_node_1] -> combine Phi_bar_psi_e/1(Phi_bar_psi_e_node_1)
  [V_Phi_Rei_squ_2p_vec] -> cal Phi_psi_e agent 2/9(V_Phi_Rei_squ_2p_vec)
  [theta_sigma_bar_w_tilt_2_vec] -> cal sigma_bar_w_hat agent 5/4(theta_sigma_bar_w_tilt_2_vec)
  Constant489/1 -> cal Fi_S agent 3/2(Ji)
  [V_Phi_Rei_squ_2p_vec] -> cal Phi_bar_psi_e agent 3/12(V_Phi_Rei_squ_2p_vec)
  Demux137/2 -> d2_sigma_bar_w_est_4/2
  cal theta_sigma_bar_w_tilt agent 3/1(theta_sigma_bar_w_tilt_1_3) -> [theta_sigma_bar_w_tilt_1_3]
  [dw_hat_vec] -> cal taui agent 1/7(dw_hat_vec)
  [Qi_vec] -> Qi dynam agent 5/1(Qi_vec)
  cal Phi_psi_e agent 3/1(Phi_psi_e_node_3) -> [Phi_psi_e_node_3]
  cal d_theta_hat/2(d_dui_hat) -> Integrator3/1
  [Si_vec] -> cal theta_Si_beta_w agent 2/4(Si_vec)
  Integrator28/1 -> [Qi_3]
  Constant544/1 -> cal S_bar agent 5/2(gamma0)
  [theta_Si_beta_w_2_vec] -> cal taui agent 1/10(theta_Si_beta_w_2_vec)
  Interpreted MATLAB Function112/1 -> trans to column114/1(x)
  Constant469/1 -> cal Phi_bar_psi_e agent 3/6(eps_s_bar_div_pi)
  Constant415/1 -> Mux208/2
  cal Fi_S agent 1/1(Fi_S_1) -> [Fi_S_1]
  Constant528/1 -> cal taui agent 2/2(c_w_2)
  Constant605/1 -> cal Phi_psi_e agent 5/4(thr_p_plus_1)
  [V_Phi_Rei_div_pi_vec] -> choose ksi_est_err 54/1(x)
  Constant548/1 -> cal Phi_psi_e agent 4/2(beta_Phi_2)
  Constant545/1 -> cal Phi_psi_e agent 1/3(gamma0)
  [Si_vec] -> cal taui agent 2/6(Si_vec)
  Constant382/1 -> Product9/2
  [V_Phi_Rei_squ_p_plus_1_vec] -> cal S_bar agent 4/6(V_Phi_Rei_squ_p_plus_1_vec)
  [Si_squ_beta_w_2_node_3] -> combine Si_squ_beta_w_2/3(Si_squ_beta_w_2_node_3)
  [V_Phi_Rei_squ_2p_vec] -> cal Phi_psi_e agent 5/9(V_Phi_Rei_squ_2p_vec)
  Interpreted MATLAB Function104/1 -> trans to column106/1(x)
  [wi_3] -> combine dwi/3(wi_3)
  cal sigma_bar_w_hat agent 2/1(d_sigma_bar_w_hat_2) -> sigma_bar_w_hat Integrator 2/1
  [V_Phi_Rei_squ_p_plus_1_vec] -> cal Phi_psi_e agent 3/8(V_Phi_Rei_squ_p_plus_1_vec)
  [Qi_4] -> combine Qi Ri/4(Qi_4)
  Memory23/1 -> [theta_Si_beta_w_1_vec]
  Constant366/1 -> Mux165/3
  Constant501/1 -> Mux196/3
  [theta_Si_beta_w_2_vec] -> cal taui agent 2/10(theta_Si_beta_w_2_vec)
  combine V_Phi_Rei_squ_p_plus_1/1(V_Phi_Rei_squ_p_plus_1_vec) -> Memory10/1
  [V_Phi_Rei_squ_p_min_1_node_4] -> combine V_Phi_Rei_squ_p_min_1/4(V_Phi_Rei_squ_p_min_1_node_4)
  sigma_bar_w_hat Integrator 2/1 -> [sigma_bar_w_hat_2]
  choose ui agent 2/1(y) -> Add27/2
  [wei_vec] -> cal Fi_S agent 3/5(wei_vec)
  Interpreted MATLAB Function81/1 -> trans to column81/1(x)
  Constant585/1 -> cal Phi_psi_e agent 3/2(beta_Phi_2)
  [ui_squ_2_node_1] -> cal sig1/1(x)
  combine V_Phi_Rei_squ_p_min_1/1(V_Phi_Rei_squ_p_min_1_vec) -> Memory25/1
  Constant475/1 -> cal Phi_bar_psi_e agent 4/6(eps_s_bar_div_pi)
  [ui_vec] -> choose ui agent 4/1(x)
  Demux123/2 -> Mux177/2
  choose ksi_est_err 53/1(y) -> cal abs 73/1(x)
  cal sig10/1(z) -> [ui_sig_4_node_2]
  Constant319/1 -> cal d_theta_hat3/1(c1)
  Add24/1 -> Mux141/2
  Constant327/1 -> Mux157/3
  [dw_vec] -> wi dynam agent 3/4(dw_vec)
  Constant318/1 -> Mux153/2
  Integrator48/1 -> [sigma_w_3]
  Constant348/1 -> Mux160/3
  [dw_vec] -> wi dynam agent 4/4(dw_vec)
  cal divide pi/1(y) -> [V_Phi_Rei_div_pi_vec]
  [dw_vec] -> wi dynam agent 2/4(dw_vec)
  [dw_vec] -> wi dynam agent 1/4(dw_vec)
  Constant533/1 -> cal S_bar agent 5/1(cS0)
  combine tau1/1(dw_vec) -> [dw_vec]
  [ui_sig_5_node_4] -> cal d_theta_hat3/9(ui_sig_5)
  [Rei_vec] -> cal wei agent 3/2(Rei_vec)
  Demux119/1 -> Mux178/1
  [theta_sigma_bar_w_tilt_2_vec] -> cal sigma_bar_w_hat agent 2/4(theta_sigma_bar_w_tilt_2_vec)
  Mux198/1 -> Interpreted MATLAB Function106/1
  [sigma_bar_w_hat_2] -> combine sigma_bar_w_hat/2(sigma_bar_w_hat_2)
  Constant581/1 -> cal Phi_psi_e agent 2/4(thr_p_plus_1)
  [theta_sigma_bar_w_tilt_2_5] -> combine theta_sigma_bar_w_tilt/10(theta_sigma_bar_w_tilt_2_5)
  Mux206/1 -> Interpreted MATLAB Function114/1
  Memory9/1 -> [Phi_bar_psi_e_vec]
  cal sigma_bar_w_hat agent 4/1(d_sigma_bar_w_hat_4) -> sigma_bar_w_hat Integrator 4/1
  Demux132/3 -> d_sigma_bar_w_est_1/3
  [V_Phi_Rei_squ_p_plus_1_vec] -> cal Phi_psi_e agent 2/8(V_Phi_Rei_squ_p_plus_1_vec)
  [taui_vec] -> cal d_sigma_w agent 2/4(taui_vec)
  Integrator9/1 -> Display132/1, Demux102/1, [d2_ui_hat_node_3]
  [sigma_bar_w_vec] -> cal d_sigma_w agent 4/5(sigma_w_bar_vec)
  Constant423/1 -> Mux207/2
  Constant445/1 -> cal dw_hat agent 1/1(h3w)
  Memory19/1 -> [Si_vec]
  [theta_sigma_bar_w_tilt_1_vec] -> cal sigma_bar_w_hat agent 2/3(theta_sigma_bar_w_tilt_1_vec)
  [theta_sigma_bar_w_tilt_2_vec] -> cal sigma_bar_w_hat agent 4/4(theta_sigma_bar_w_tilt_2_vec)
  cal differentiator d_sigma_bar_w_hat agent 2/1(Out1) -> Display107/1, [sigma_bar_w_est_2]
  Constant602/1 -> Mux213/3
  cal differentiator d_sigma_bar_w_hat agent 4/1(Out1) -> Display117/1, [sigma_bar_w_est_4]
  Demux112/3 -> wci_node_3/3
  Integrator47/1 -> [sigma_w_2]
  Constant429/1 -> Mux199/3
  choose ui agent 3/1(y) -> Add13/2
  trans to column108/1(y) -> [sigma_bar_w_tilt_squ_1_1], Display171/1
  cal wci dwci agent 1/1(wci) -> Display142/1, Demux105/1, [wci_node_1]
  sigma_bar_w_hat Integrator 4/1 -> [sigma_bar_w_hat_4]
  [d_sigma_bar_w_vec] -> cal dw_hat agent 1/3(d_sigma_bar_w_vec)
  [wi_vec] -> cal wei agent 4/1(wi_vec)
  cal abs 69/1(y) -> Mux204/1
  cal abs 70/1(y) -> Mux203/1
  Constant378/1 -> Product6/2
  cal theta_sigma_bar_w_tilt agent 2/1(theta_sigma_bar_w_tilt_1_2) -> [theta_sigma_bar_w_tilt_1_2]
  cal abs 66/1(y) -> Mux200/1
  [d_sigma_bar_w_vec] -> cal sigma_bar_w_hat agent 5/5(d_sigma_bar_w_vec)
  [taui_vec] -> cal d_sigma_w agent 4/4(taui_vec)
  [sigma_bar_w_hat_1] -> combine sigma_bar_w_hat/1(sigma_bar_w_hat_1)
  Integrator27/1 -> [Qi_2]
  Memory4/1 -> [Ri_vec]
  Demux131/2 -> d2_sigma_bar_w_est_1/2
  Mux179/1 -> Scope14/3
  [sigma_bar_w_tilt_squ_1_4] -> cal theta_sigma_bar_w_tilt agent 4/2(sigma_bar_w_tilt_squ_1_4)
  Constant313/1 -> Add29/1
  [sigma_w_4] -> combine sigma_w/4(sigma_w_4)
  combine d_sigma_bar_v_est1/1(d_sigma_bar_w_vec) -> [d_sigma_bar_w_vec]
  [V_Phi_Rei_squ_p_min_1_node_3] -> combine V_Phi_Rei_squ_p_min_1/3(V_Phi_Rei_squ_p_min_1_node_3)
  Abs27/1 -> Mux161/1
  Constant443/1 -> cal sigma_bar_w_hat agent 5/2(h2w)
  [d2uihat_vec] -> cal wci dwci agent 1/3(d2uihat_vec)
  Mux176/1 -> Scope13/1
  Constant456/1 -> cal dw_hat agent 5/1(h3w)
  sigma_bar_w_hat Integrator 1/1 -> [sigma_bar_w_hat_1]
  [sigma_bar_w_tilt_squ_1_3] -> cal theta_sigma_bar_w_tilt agent 3/2(sigma_bar_w_tilt_squ_1_3)
  cal sig5/1(z) -> [ui_sig_5_node_1]
  Mux203/1 -> Interpreted MATLAB Function110/1
  [wi_vec] -> Qi dynam agent 2/2(wi_vec)
  Constant413/1 -> cal d_sigma_w agent 1/2(Ji)
  [dw_hat_2] -> combine dw_hat/2(dw_hat_2)
  [dw_vec] -> cal error dw_tilt/1(dw_vec)
  [d_sigma_bar_w_est_3] -> combine d_sigma_bar_v_est1/3(d_sigma_bar_w_est_3)
  cal d_sigma_w agent 5/1(d_sigma_w_5) -> Integrator50/1
  [sigma_bar_w_hat_vec] -> cal dw_hat agent 2/4(sigma_bar_w_hat_vec)
  Constant452/1 -> cal dw_hat agent 1/2(Ji)
  cal theta_sigma_bar_w_tilt agent 1/1(theta_sigma_bar_w_tilt_1_1) -> [theta_sigma_bar_w_tilt_1_1]
  Memory25/1 -> [V_Phi_Rei_squ_p_min_1_vec]
  Constant446/1 -> cal dw_hat agent 2/1(h3w)
  [Qci_5] -> combine Qci Rci/5(Qci_5)
  Mux200/1 -> Interpreted MATLAB Function108/1
  cal abs 71/1(y) -> Mux207/1
  [wi_vec] -> cal d_sigma_w agent 2/3(wi_vec)
  [sigma_bar_w_hat_vec] -> cal dw_hat agent 5/4(sigma_bar_w_hat_vec)
  [sigma_bar_w_tilt_vec] -> choose ksi_est_err 45/1(x)
  Constant448/1 -> cal dw_hat agent 3/1(h3w)
  Demux131/3 -> d2_sigma_bar_w_est_1/3
  [sigma_bar_w_tilt_vec] -> cal theta_sigma_bar_w_tilt agent 1/4(sigma_bar_w_tilt_vec)
  Add11/1 -> Mux215/2
  [d2uihat_vec] -> cal wci dwci agent 4/3(d2uihat_vec)
  Qi dynam agent 1/1(dQi_1) -> Integrator26/1
  [taui_vec] -> cal d_sigma_w agent 1/4(taui_vec)
  Demux136/2 -> d_sigma_bar_w_est_3/2
  cal differentiator d_sigma_bar_w_hat agent 4/3(Out3) -> Demux137/1, [d2_sigma_bar_w_est_4], Display166/1
  Demux141/2 -> d_sigma_bar_w_est_5/2
  choose ui agent 4/1(y) -> Add15/2
  [dw_hat_4] -> combine dw_hat/4(dw_hat_4)
  [Qei_vec] -> Qei dynam agent 3/1(Qei_vec)
  Demux138/2 -> d_sigma_bar_w_est_4/2
  [sigma_bar_w_tilt_vec] -> cal theta_sigma_bar_w_tilt agent 2/4(sigma_bar_w_tilt_vec)
  Demux140/3 -> d2_sigma_bar_w_est_5/3
  Constant376/1 -> Add16/2
  Constant408/1 -> Mux200/3
  Constant638/1 -> cal d_theta_hat1/4(chi_t)
  [d_sigma_bar_w_est_2] -> combine d_sigma_bar_v_est1/2(d_sigma_bar_w_est_2)
  cal differentiator d_sigma_bar_w_hat agent 5/1(Out1) -> Display169/1, [sigma_bar_w_est_5]
  Memory10/1 -> [V_Phi_Rei_squ_p_plus_1_vec]
  Mux156/1 -> Interpreted MATLAB Function79/1
  [sigma_bar_w_vec] -> cal differentiator d_sigma_bar_w_hat agent 5/1(x)
  [ui_squ_6_node_5] -> cal sig29/1(x)
  Constant438/1 -> cal sigma_bar_w_hat agent 3/1(h1w)
  Mux148/1 -> Interpreted MATLAB Function71/1
  choose ksi_est_err 46/1(y) -> cal abs 66/1(x)
  trans to column120/1(y) -> [Si_squ_beta_w_1_node_4], Display161/1
  [Qei_vec] -> cal Rei agent 5/1(Qei_vec)
  choose ksi_est_err 51/1(y) -> cal abs 71/1(x)
  Demux128/3 -> ui_tilt_node_5/3
  [wi_vec] -> wi dynam agent 2/2(wi_vec)
  trans to column114/1(y) -> [sigma_bar_w_tilt_squ_2_5], Display111/1
  Constant430/1 -> Mux198/2
  cal abs 73/1(y) -> Mux205/1
  Mux208/1 -> Interpreted MATLAB Function115/1
  Constant458/1 -> cal d_sigma_w agent 4/1(h3w)
  [sigma_bar_w_tilt_squ_1_5] -> cal theta_sigma_bar_w_tilt agent 5/2(sigma_bar_w_tilt_squ_1_5)
  cal d_sigma_w agent 3/1(d_sigma_w_3) -> Integrator48/1
  [sigma_bar_w_tilt_vec] -> cal theta_sigma_bar_w_tilt agent 3/4(sigma_bar_w_tilt_vec)
  Mux186/1 -> Scope1/2
  [Qei_vec] -> cal Qci agent 4/2(Qei_vec)
  [dw_hat_3] -> combine dw_hat/3(dw_hat_3)
  [sigma_bar_w_tilt_squ_2_2] -> cal theta_sigma_bar_w_tilt agent 2/3(sigma_bar_w_tilt_squ_2_2)
  Interpreted MATLAB Function108/1 -> trans to column109/1(x)
  [d_sigma_bar_w_vec] -> cal sigma_bar_w_hat agent 2/5(d_sigma_bar_w_vec)
  [sigma_bar_w_hat_vec] -> cal dw_hat agent 4/4(sigma_bar_w_hat_vec)
  combine sigma_w/1(sigma_w_vec) -> [sigma_w_vec]
  [ui_tilt_node_5] -> Abs26/1
  cal sigma_bar_w_hat agent 1/1(d_sigma_bar_w_hat_1) -> sigma_bar_w_hat Integrator 1/1
  Constant321/1 -> Add16/1
  [V_Phi_Rei_div_pi_vec] -> cal S_bar agent 5/5(V_Phi_Rei_div_pi_vec)
  [sigma_bar_w_vec] -> cal combine sigma_bar_w_tilt/1(sigma_bar_w_vec)
  [sigma_bar_w_vec] -> cal differentiator d_sigma_bar_w_hat agent 4/1(x)
  [sigma_bar_w_hat_5] -> combine sigma_bar_w_hat/5(sigma_bar_w_hat_5)
  [d_sigma_bar_w_vec] -> cal sigma_bar_w_hat agent 4/5(d_sigma_bar_w_vec)
  wi dynam agent 1/1(dwi_1) -> Integrator21/1
  [Phi_bar_psi_e_node_3] -> combine Phi_bar_psi_e/3(Phi_bar_psi_e_node_3)
  Demux137/3 -> d2_sigma_bar_w_est_4/3
  cal abs 68/1(y) -> Mux208/1
  Constant434/1 -> cal sigma_bar_w_hat agent 1/2(h2w)
  cal abs 65/1(y) -> Mux206/1
  [Rci_vec] -> cal wci dwci agent 4/4(Rci_mat)
  Constant379/1 -> Product7/2
  Mux181/1 -> Scope14/1
  Demux135/3 -> d2_sigma_bar_w_est_3/3
  Constant399/1 -> cal S_bar agent 3/3(thr_p_plus_1)
  [ui_sig_6_node_3] -> cal d_theta_hat2/10(ui_sig_6)
  [theta_sigma_bar_w_tilt_1_1] -> combine theta_sigma_bar_w_tilt/1(theta_sigma_bar_w_tilt_1_1)
  cal abs 92/1(y) -> Mux165/1
  [tau_5] -> combine tau/5(tau_5)
  cal taui agent 1/1(tau_1) -> [tau_1]
  Constant356/1 -> Mux163/3
  Demux100/1 -> d2_ui_hat_node_1/1
  Interpreted MATLAB Function105/1 -> trans to column89/1(x)
  cal S_bar agent 2/1(S_bar_node_2) -> [S_bar_node_2]
  Constant335/1 -> Mux188/2
  [V_Phi_Rei_squ_p_min_1_node_2] -> combine V_Phi_Rei_squ_p_min_1/2(V_Phi_Rei_squ_p_min_1_node_2)
  Constant311/1 -> Mux169/3
  Constant411/1 -> Mux180/2
  cal abs 91/1(y) -> Mux180/1
  Demux129/2 -> d_ui_hat_node_3/2
  Constant412/1 -> cal theta_sigma_bar_w_tilt agent 3/1(alfa_theta_obs_w)
  Constant632/1 -> Mux158/3
  [V_Phi_Rei_div_pi_vec] -> choose ksi_est_err 70/1(x)
  trans to column83/1(y) -> [V_Phi_Rei_squ_p_plus_1_node_2], Display98/1
  [ui_tilt_node_4] -> cal sig20/2(y)
  [V_Phi_Rei_div_pi_vec] -> cal S_bar agent 2/5(V_Phi_Rei_div_pi_vec)
  cal differentiator d_sigma_bar_w_hat agent 3/2(Out2) -> Demux136/1, [d_sigma_bar_w_est_3], Display115/1
  [V_Phi_Rei_squ_2p_node_2] -> combine V_Phi_Rei_squ_2p/2(V_Phi_Rei_squ_2p_node_2)
  Integrator7/1 -> Display130/1, [ui_hat_node_3]
  [dw_3] -> combine tau1/3(dw_3)
  Constant421/1 -> Mux203/3
  Interpreted MATLAB Function103/1 -> trans to column104/1(x)
  [V_Phi_Rei_squ_2p_node_3] -> combine V_Phi_Rei_squ_2p/3(V_Phi_Rei_squ_2p_node_3)
  Demux102/3 -> d2_ui_hat_node_3/3
  cal wci dwci agent 4/1(wci) -> Display148/1, Demux114/1, [wci_node_4]
  Constant599/1 -> cal S_bar agent 1/2(gamma0)
  [wei_vec] -> cal Phi_bar_psi_e agent 4/7(wei_vec)
  Constant610/1 -> cal S_bar agent 1/3(thr_p_plus_1)
  Demux130/3 -> d_ui_hat_node_1/3
  [wei_vec] -> cal S_bar agent 1/4(wei_vec)
  [V_Phi_Rei_squ_p_plus_1_node_1] -> combine V_Phi_Rei_squ_p_plus_1/1(V_Phi_Rei_squ_p_plus_1_node_1)
  Constant333/1 -> cal S_bar agent 2/2(gamma0)
  [V_Phi_Rei_squ_p_plus_1_node_5] -> combine V_Phi_Rei_squ_p_plus_1/5(V_Phi_Rei_squ_p_plus_1_node_5)
  Memory6/1 -> [wei_vec]
  trans to column111/1(y) -> [sigma_bar_w_tilt_squ_1_3], Display105/1
  Mux147/1 -> Interpreted MATLAB Function72/1
  [V_Phi_Rei_squ_p_plus_1_node_4] -> combine V_Phi_Rei_squ_p_plus_1/4(V_Phi_Rei_squ_p_plus_1_node_4)
  [ui_tilt_node_2] -> Abs11/1
  Mux163/1 -> Interpreted MATLAB Function86/1
  [taui_vec] -> cal d_sigma_w agent 3/4(taui_vec)
  [sigma_bar_w_tilt_vec] -> choose ksi_est_err 43/1(x)
  Demux118/1 -> Mux171/2
  cal dw_hat agent 1/1(dw_hat_1) -> [dw_hat_1]
  [ui_tilt_node_5] -> Abs29/1
  Mux136/1 -> Interpreted MATLAB Function61/1
  [Rci_vec] -> cal wci dwci agent 1/4(Rci_mat)
  [Si_vec] -> choose ksi_est_err 61/1(x)
  [ui_squ_1_node_5] -> cal sig26/1(x)
  Constant331/1 -> Mux155/2
  cal differentiator d_sigma_bar_w_hat agent 2/2(Out2) -> Demux134/1, [d_sigma_bar_w_est_2], Display110/1
  Constant635/1 -> Mux144/3
  cal theta_Si_beta_w agent 1/2(theta_Si_beta_w_2_node_1) -> [theta_Si_beta_w_2_node_1]
  Demux125/3 -> Mux179/2
  [ui_sig_2_node_5] -> cal d_theta_hat4/6(ui_sig_2)
  Mux177/1 -> Scope13/2
  cal differentiator d_sigma_bar_w_hat agent 5/2(Out2) -> Demux141/1, [d_sigma_bar_w_est_5], Display167/1
  Constant490/1 -> cal Fi_S agent 4/1(cS0)
  [tsim] -> generate angular rate disturbance agent 1/4(t)
  [tsim] -> generate angular rate disturbance agent 2/4(t)
  Constant561/1 -> generate angular rate disturbance agent 2/1(dw_aa_t)
  [Qei_vec] -> cal Qci agent 3/2(Qei_vec)
  generate angular rate disturbance agent 2/1(dw_2) -> [dw_2]
  Constant466/1 -> cal S_bar agent 4/2(gamma0)
  choose ksi_est_err 73/1(y) -> cal abs 93/1(x)
  [sigma_bar_w_tilt_vec] -> choose ksi_est_err 50/1(x)
  Mux166/1 -> Interpreted MATLAB Function90/1
  [ui_sig_6_node_5] -> cal d_theta_hat4/10(ui_sig_6)
  cal sig2/1(z) -> [ui_sig_3_node_1]
  Interpreted MATLAB Function90/1 -> trans to column92/1(x)
  Constant431/1 -> Mux198/3
  trans to column89/1(y) -> [V_Phi_Rei_squ_p_plus_1_node_3], Display118/1
  trans to column90/1(y) -> [V_Phi_Rei_squ_2p_node_3], Display119/1
  Constant515/1 -> cal theta_Si_beta_w agent 4/1(mu_c_theta)
  [V_Phi_Rei_div_pi_vec] -> cal S_bar agent 4/5(V_Phi_Rei_div_pi_vec)
  [V_Phi_Rei_div_pi_vec] -> choose ksi_est_err 72/1(x)
  [d2_ui_hat_node_3] -> cal d_theta_hat2/12(d2ui_hat)
  Constant570/1 -> generate angular rate disturbance agent 5/1(dw_aa_t)
  Mux165/1 -> Interpreted MATLAB Function89/1
  cal sig15/1(z) -> [ui_sig_2_node_3]
  [d2_ui_hat_node_5] -> combine duihat d2uihat/10(d2_ui_hat_node_5)
  cal abs 64/1(y) -> Mux198/1
  Mux161/1 -> Interpreted MATLAB Function85/1
  Abs9/1 -> Mux144/1
  Demux133/1 -> d2_sigma_bar_w_est_2/1
  wi dynam agent 5/1(dwi_5) -> Integrator25/1
  Interpreted MATLAB Function78/1 -> trans to column77/1(x)
  [theta_Si_beta_w_1_node_2] -> combine theta_Si_beta_w_1/2(theta_Si_beta_w_1_node_2)
  [V_Phi_Rei_squ_2p_vec] -> cal Phi_bar_psi_e agent 4/12(V_Phi_Rei_squ_2p_vec)
  [theta_sigma_bar_w_tilt_2_vec] -> cal sigma_bar_w_hat agent 1/4(theta_sigma_bar_w_tilt_2_vec)
  [Fi_S_4] -> combine Fi_S/4(Fi_S_4)
  Interpreted MATLAB Function72/1 -> trans to column72/1(x)
  [ui_sig_2_node_3] -> cal d_theta_hat2/6(ui_sig_2)
  [Fi_S_5] -> combine Fi_S/5(Fi_S_5)
  [ui_squ_4_node_2] -> cal sig10/1(x)
  [V_Phi_Rei_squ_p_plus_1_vec] -> cal Phi_bar_psi_e agent 4/11(V_Phi_Rei_squ_p_plus_1_vec)
  combine Fi_S/1(Fi_S_vec) -> Memory20/1
  [wei_vec] -> cal Phi_bar_psi_e agent 3/7(wei_vec)
  Constant600/1 -> cal d_theta_hat/3(c3)
  [wi_vec] -> cal Fi_S agent 5/3(wi_vec)
  [sigma_bar_w_hat_vec] -> cal dw_hat agent 1/4(sigma_bar_w_hat_vec)
  Constant493/1 -> cal Fi_S agent 5/2(Ji)
  Constant488/1 -> Mux167/2
  Constant468/1 -> cal Phi_bar_psi_e agent 3/5(gamma0)
  Constant492/1 -> cal Fi_S agent 5/1(cS0)
  [V_Phi_Rei_div_pi_vec] -> cal Phi_bar_psi_e agent 5/9(V_Phi_Rei_div_pi_vec)
  Constant472/1 -> cal Phi_bar_psi_e agent 4/3(beta_Phi_2)
  [V_Phi_Rei_div_pi_vec] -> choose ksi_est_err 73/1(x)
  [wei_vec] -> cal Fi_S agent 4/5(wei_vec)
  cal Si agent 1/1(Si_1) -> [Si_1]
  Demux141/3 -> d_sigma_bar_w_est_5/3
  Constant414/1 -> Mux201/3
  [wci_vec] -> cal Fi_S agent 4/4(wci_vec)
  Interpreted MATLAB Function116/1 -> trans to column105/1(x)
  [Phi_bar_psi_e_vec] -> cal Fi_S agent 3/8(Phi_bar_psi_e_vec)
  Demux108/3 -> ui_tilt_node_1/3
  [Qi_3] -> combine Qi Ri/3(Qi_3)
  choose ksi_est_err 57/1(y) -> cal abs 77/1(x)
  [V_Phi_Rei_div_pi_vec] -> cal Phi_psi_e agent 3/7(V_Phi_Rei_div_pi_vec)
  Constant491/1 -> cal Fi_S agent 4/2(Ji)
  [Rei_vec] -> cal Fi_S agent 2/7(Rei_vec)
  Constant303/1 -> Mux146/2
  combine Qi Ri/2(Ri_vec) -> Memory4/1
  cal sig18/1(z) -> [ui_sig_4_node_4]
  Constant485/1 -> cal Fi_S agent 2/1(cS0)
  [wci_node_5] -> combine wci dwci/5(wci_node_5)
  Constant441/1 -> cal sigma_bar_w_hat agent 4/2(h2w)
  cal Fi_S agent 2/1(Fi_S_2) -> [Fi_S_2]
  [wei_vec] -> cal Fi_S agent 2/5(wei_vec)
  Memory7/1 -> [Qei_vec]
  Interpreted MATLAB Function86/1 -> trans to column86/1(x)
  Constant353/1 -> cal d_theta_hat4/3(c3)
  [S_bar_vec] -> cal Phi_bar_psi_e agent 1/8(S_bar_vec)
  Abs5/1 -> Mux138/1
  [V_Phi_Rei_squ_p_plus_1_vec] -> cal S_bar agent 2/6(V_Phi_Rei_squ_p_plus_1_vec)
  Interpreted MATLAB Function107/1 -> trans to column108/1(x)
  [Phi_bar_psi_e_vec] -> cal Fi_S agent 2/8(Phi_bar_psi_e_vec)
  [wci_vec] -> cal Fi_S agent 2/4(wci_vec)
  Demux111/3 -> ui_tilt_node_3/3
  combine sigma_bar_w_hat/1(sigma_bar_w_hat_vec) -> [sigma_bar_w_hat_vec]
  [wi_vec] -> cal Fi_S agent 1/3(wi_vec)
  [ui_hat_node_3] -> Demux122/1
  Constant424/1 -> cal theta_sigma_bar_w_tilt agent 5/1(alfa_theta_obs_w)
  Constant427/1 -> Mux205/2
  [wci_vec] -> cal Fi_S agent 1/4(wci_vec)
  cal Phi_bar_psi_e agent 5/1(Phi_bar_psi_e_node_5) -> [Phi_bar_psi_e_node_5]
  Constant478/1 -> cal Phi_bar_psi_e agent 5/2(beta_Phi_1)
  [wi_vec] -> cal wei agent 3/1(wi_vec)
  cal taui agent 3/1(tau_3) -> [tau_3]
  Constant484/1 -> cal Fi_S agent 1/2(Ji)
  Constant483/1 -> cal Fi_S agent 1/1(cS0)
  [S_bar_vec] -> cal Phi_psi_e agent 2/6(S_bar_vec)
  cal theta_sigma_bar_w_tilt agent 1/2(theta_sigma_bar_w_tilt_2_1) -> [theta_sigma_bar_w_tilt_2_1]
  [dwci_node_1] -> combine wci dwci/6(dwci_node_1)
  Demux110/2 -> ui_tilt_node_2/2
  Abs3/1 -> Mux215/1
  [V_Phi_Rei_div_pi_vec] -> cal Phi_bar_psi_e agent 4/9(V_Phi_Rei_div_pi_vec)
  [S_bar_vec] -> cal Phi_bar_psi_e agent 3/8(S_bar_vec)
  [S_bar_vec] -> cal Phi_bar_psi_e agent 4/8(S_bar_vec)
  Constant343/1 -> Mux155/3
  Constant473/1 -> cal Phi_bar_psi_e agent 4/4(thr_p_plus_1)
  Demux109/1 -> dwci_node_2/1
  [d_sigma_bar_w_vec] -> cal sigma_bar_w_hat agent 1/5(d_sigma_bar_w_vec)
  Constant465/1 -> cal Phi_bar_psi_e agent 3/3(beta_Phi_2)
  [ui_tilt_node_3] -> Abs16/1
  Demux134/2 -> d_sigma_bar_w_est_2/2
  Constant467/1 -> cal Phi_bar_psi_e agent 3/4(thr_p_plus_1)
  [V_Phi_Rei_div_pi_vec] -> cal Phi_bar_psi_e agent 3/9(V_Phi_Rei_div_pi_vec)
  Demux101/3 -> d2_ui_hat_node_2/3
  Mux182/1 -> Scope14/2
  Demux140/1 -> d2_sigma_bar_w_est_5/1
  Constant606/1 -> cal Phi_psi_e agent 5/5(eps_s_bar_div_pi)
  [V_Phi_Rei_squ_p_plus_1_vec] -> cal Phi_bar_psi_e agent 3/11(V_Phi_Rei_squ_p_plus_1_vec)
  cal abs 72/1(y) -> Mux147/1
  [theta_sigma_bar_w_tilt_1_4] -> combine theta_sigma_bar_w_tilt/4(theta_sigma_bar_w_tilt_1_4)
  [wei_vec] -> cal Fi_S agent 5/5(wei_vec)
  trans to column79/1(y) -> [ui_squ_3_node_4]
  Mux178/1 -> Scope1/1
  Demux133/2 -> d2_sigma_bar_w_est_2/2
  cal d_theta_hat4/2(d_dui_hat) -> Integrator14/1
  Constant418/1 -> cal theta_sigma_bar_w_tilt agent 4/1(alfa_theta_obs_w)
  [V_Phi_Rei_4] -> combine Qci Rci1/4(V_Phi_Rei_4)
  Interpreted MATLAB Function106/1 -> trans to column107/1(x)
  Demux103/2 -> d2_ui_hat_node_4/2
  [V_Phi_Rei_div_pi_vec] -> cal Phi_bar_psi_e agent 2/9(V_Phi_Rei_div_pi_vec)
  Constant393/1 -> cal Phi_bar_psi_e agent 1/5(gamma0)
  [ui_squ_3_node_3] -> cal sig16/1(x)
  Demux117/3 -> dwci_node_5/3
  trans to column72/1(y) -> [V_Phi_Rei_squ_2p_node_1], Display97/1
  Demux/3 -> Mux173/1
  [Qi_vec] -> cal Ri agent 5/1(Qi_vec)
  cal differentiator d_sigma_bar_w_hat agent 1/2(Out2) -> Demux132/1, [d_sigma_bar_w_est_1], Display104/1
  choose ksi_est_err 49/1(y) -> cal abs 69/1(x)
  [wei_vec] -> Qei dynam agent 3/2(wei_vec)
  Constant389/1 -> cal Phi_bar_psi_e agent 1/1(pp0)
  combine Phi_bar_psi_e/1(Phi_bar_psi_e_vec) -> Memory9/1
  [ui_squ_3_node_1] -> cal sig2/1(x)
  Constant341/1 -> Mux192/2
  Constant322/1 -> cal S_bar agent 2/1(cS0)
  Mux192/1 -> Interpreted MATLAB Function99/1
  [dw_4] -> combine tau1/4(dw_4)
  Constant639/1 -> Mux149/2
  [Phi_bar_psi_e_node_4] -> combine Phi_bar_psi_e/4(Phi_bar_psi_e_node_4)
  Mux155/1 -> Interpreted MATLAB Function76/1
  [dw_1] -> combine tau1/1(dw_1)
  cal abs 78/1(y) -> Mux192/1
  [sigma_bar_w_vec] -> cal d_sigma_w agent 2/5(sigma_w_bar_vec)
  [Qi_vec] -> cal Qci agent 4/1(Qi_vec)
  Mux167/1 -> Interpreted MATLAB Function91/1
  Constant549/1 -> cal Phi_psi_e agent 5/2(beta_Phi_2)
  choose ksi_est_err 56/1(y) -> cal abs 76/1(x)
  [wei_5] -> combine wei Qei Rei/5(wei_5)
  Mux187/1 -> Interpreted MATLAB Function95/1
  [wci_vec] -> cal wei agent 3/3(wci_vec)
  Constant338/1 -> Mux189/3
  trans to column107/1(y) -> [sigma_bar_w_tilt_squ_2_1], Display170/1
  [Rei_vec] -> cal Fi_S agent 5/7(Rei_vec)
  cal abs 76/1(y) -> Mux189/1
  Mux190/1 -> Interpreted MATLAB Function98/1
  Interpreted MATLAB Function96/1 -> trans to column97/1(x)
  cal d_theta_hat/1(d_ui_hat) -> Integrator2/1
  Demux134/3 -> d_sigma_bar_w_est_2/3
  Constant576/1 -> cal Phi_psi_e agent 1/5(eps_s_bar_div_pi)
  [V_Phi_Rei_div_pi_vec] -> choose ksi_est_err 56/1(x)
  Demux139/2 -> d_ui_hat_node_2/2
  trans to column98/1(y) -> [V_Phi_Rei_squ_p_min_1_node_3], Display141/1
  cal abs 93/1(y) -> Mux167/1
  Demux128/1 -> ui_tilt_node_5/1
  Constant337/1 -> Mux189/2
  [d_sigma_bar_w_vec] -> cal dw_hat agent 5/3(d_sigma_bar_w_vec)
  Mux191/1 -> Interpreted MATLAB Function116/1
  Demux137/1 -> d2_sigma_bar_w_est_4/1
  Demux99/2 -> d_ui_hat_node_5/2
  Demux140/2 -> d2_sigma_bar_w_est_5/2
  Constant336/1 -> Mux188/3
  Mux188/1 -> Interpreted MATLAB Function96/1
  choose ksi_est_err 55/1(y) -> cal abs 75/1(x)
  Constant422/1 -> Mux180/3
  [Si_4] -> combine Si/4(Si_4)
  Constant583/1 -> cal Phi_psi_e agent 3/3(gamma0)
  [Phi_psi_e_vec] -> cal Si agent 5/3(Phi_psi_e_vec)
  Demux135/1 -> d2_sigma_bar_w_est_3/1
  [V_Phi_Rei_squ_2p_vec] -> cal Phi_psi_e agent 1/9(V_Phi_Rei_squ_2p_vec)
  cal Si agent 5/1(Si_5) -> [Si_5]
  Integrator29/1 -> [Qi_4]
  [wei_vec] -> cal Si agent 5/2(wei_vec)
  [theta_sigma_bar_w_tilt_2_vec] -> cal sigma_bar_w_hat agent 3/4(theta_sigma_bar_w_tilt_2_vec)
  cal S_bar agent 1/1(S_bar_node_1) -> [S_bar_node_1]
  [ui_tilt_node_2] -> Abs7/1
  [Qei_1] -> combine wei Qei Rei/6(Qei_1)
  [wei_vec] -> cal Si agent 4/2(wei_vec)
  [ui_tilt_node_4] -> Abs23/1
  Constant613/1 -> cal Si agent 4/1(cS0)
  Constant439/1 -> cal sigma_bar_w_hat agent 3/2(h2w)
  [wei_vec] -> cal Si agent 2/2(wei_vec)
  [ui_sig_2_node_4] -> cal d_theta_hat3/6(ui_sig_2)
  Demux100/2 -> d2_ui_hat_node_1/2
  [wei_vec] -> cal Si agent 3/2(wei_vec)
  Demux135/2 -> d2_sigma_bar_w_est_3/2
  cal Si agent 3/1(Si_3) -> [Si_3]
  cal wci dwci agent 4/2(dwci) -> Display149/1, Demux115/1, [dwci_node_4]
  [Phi_psi_e_node_5] -> combine Phi_psi_e/5(Phi_psi_e_node_5)
  cal abs 67/1(y) -> Mux201/1
  [V_Phi_Rei_div_pi_vec] -> cal S_bar agent 1/5(V_Phi_Rei_div_pi_vec)
  [Phi_psi_e_node_4] -> combine Phi_psi_e/4(Phi_psi_e_node_4)
  [ui_sig_4_node_4] -> cal d_theta_hat3/8(ui_sig_4)
  cal Phi_psi_e agent 2/1(Phi_psi_e_node_2) -> [Phi_psi_e_node_2]
  Constant628/1 -> cal d_theta_hat1/2(c2)
  Abs11/1 -> Mux140/1
  [V_Phi_Rei_squ_p_plus_1_vec] -> cal Phi_psi_e agent 1/8(V_Phi_Rei_squ_p_plus_1_vec)
  cal sig8/1(z) -> [ui_sig_3_node_2]
  [S_bar_vec] -> cal Phi_psi_e agent 1/6(S_bar_vec)
  Demux125/1 -> Mux181/2
  [V_Phi_Rei_div_pi_vec] -> choose ksi_est_err 75/1(x)
  [ui_tilt_node_1] -> cal sig5/2(y)
  [wci_node_1] -> combine wci dwci/1(wci_node_1)
  Integrator31/1 -> [Qei_1]
  choose ksi_est_err 50/1(y) -> cal abs 70/1(x)
  Add25/1 -> Mux144/2
  [wei_vec] -> cal S_bar agent 5/4(wei_vec)
  Constant529/1 -> cal taui agent 2/3(c_w_3)
  [theta_sigma_bar_w_tilt_2_2] -> combine theta_sigma_bar_w_tilt/7(theta_sigma_bar_w_tilt_2_2)
  [ui_hat_node_4] -> Add15/1
  [Qi_vec] -> cal Ri agent 3/1(Qi_vec)
  Mux164/1 -> Interpreted MATLAB Function87/1
  Demux132/1 -> d_sigma_bar_w_est_1/1
  Constant404/1 -> Mux206/2
  sigma_bar_w_hat Integrator 3/1 -> [sigma_bar_w_hat_3]
  [Si_vec] -> cal theta_Si_beta_w agent 1/4(Si_vec)
  [wi_vec] -> cal sigma_w_bar/1(wi_vec)
  Constant426/1 -> Mux207/3
  [sigma_bar_w_tilt_vec] -> choose ksi_est_err 44/1(x)
  Constant524/1 -> cal taui agent 1/2(c_w_2)
  [Qi_vec] -> Qi dynam agent 1/1(Qi_vec)
  [Si_squ_beta_w_1_node_5] -> combine Si_squ_beta_w_1/5(Si_squ_beta_w_1_node_5)
  cal d_theta_hat3/2(d_dui_hat) -> Integrator11/1
  [wi_vec] -> cal d_sigma_w agent 1/3(wi_vec)
  Constant482/1 -> cal Phi_bar_psi_e agent 5/6(eps_s_bar_div_pi)
  Demux131/1 -> d2_sigma_bar_w_est_1/1
  [Si_squ_beta_w_1_node_1] -> combine Si_squ_beta_w_1/1(Si_squ_beta_w_1_node_1)
  [theta_Si_beta_w_1_node_5] -> combine theta_Si_beta_w_1/5(theta_Si_beta_w_1_node_5)
  [V_Phi_Rei_div_pi_vec] -> choose ksi_est_err 58/1(x)
  [Rci_vec] -> cal wci dwci agent 2/4(Rci_mat)
  [theta_Si_beta_w_1_node_4] -> combine theta_Si_beta_w_1/4(theta_Si_beta_w_1_node_4)
  Mux205/1 -> Interpreted MATLAB Function112/1
  [ui_vec] -> choose ui agent 5/1(x)
  Demux102/2 -> d2_ui_hat_node_3/2
  cal abs 61/1(y) -> Mux136/1
  [Si_squ_beta_w_2_node_1] -> combine Si_squ_beta_w_2/1(Si_squ_beta_w_2_node_1)
  Constant486/1 -> cal Fi_S agent 2/2(Ji)
  cal taui agent 2/1(tau_2) -> [tau_2]
  Constant575/1 -> cal Phi_psi_e agent 1/4(thr_p_plus_1)
  Interpreted MATLAB Function115/1 -> trans to column110/1(x)
  choose ksi_est_err 69/1(y) -> cal abs 89/1(x)
  [ui_tilt_node_2] -> cal sig6/2(y)
  Interpreted MATLAB Function117/1 -> trans to column118/1(x)
  trans to column121/1(y) -> [Si_squ_beta_w_2_node_5], Display162/1
  [theta_sigma_bar_w_tilt_1_vec] -> cal sigma_bar_w_hat agent 4/3(theta_sigma_bar_w_tilt_1_vec)
  cal abs 84/1(y) -> Mux209/1
  cal abs 89/1(y) -> Mux212/1
  [duihat_vec] -> cal wci dwci agent 5/2(duihat_vec)
  [d_sigma_bar_w_vec] -> cal dw_hat agent 4/3(d_sigma_bar_w_vec)
  Constant555/1 -> cal S_bar agent 5/3(thr_p_plus_1)
  wi dynam agent 4/1(dwi_4) -> Integrator24/1
  Qei dynam agent 4/1(dQei_4) -> Integrator34/1
  Constant449/1 -> cal d_sigma_w agent 3/1(h3w)
  cal theta_Si_beta_w agent 3/1(theta_Si_beta_w_1_node_3) -> [theta_Si_beta_w_1_node_3]
  Demux138/1 -> d_sigma_bar_w_est_4/1
  Constant496/1 -> Mux193/2
  cal Ri agent 4/1(Ri_4) -> [Ri_4]
  cal dw_hat agent 2/1(dw_hat_2) -> [dw_hat_2]
  [theta_sigma_bar_w_tilt_1_vec] -> cal sigma_bar_w_hat agent 3/3(theta_sigma_bar_w_tilt_1_vec)
  Constant481/1 -> cal Phi_bar_psi_e agent 5/5(gamma0)
  Interpreted MATLAB Function92/1 -> trans to column95/1(x)
  Constant392/1 -> cal Phi_bar_psi_e agent 1/4(thr_p_plus_1)
  cal sig1/1(z) -> [ui_sig_2_node_1]
  [wci_vec] -> cal Fi_S agent 5/4(wci_vec)
  [Si_vec] -> choose ksi_est_err 66/1(x)
  [d_sigma_bar_w_vec] -> cal dw_hat agent 3/3(d_sigma_bar_w_vec)
  [d_sigma_bar_w_est_5] -> combine d_sigma_bar_v_est1/5(d_sigma_bar_w_est_5)
  cal Ri agent 2/1(Ri_2) -> [Ri_2]
  cal d_sigma_w agent 1/1(d_sigma_w_1) -> Integrator46/1
  Constant474/1 -> cal Phi_bar_psi_e agent 4/5(gamma0)
  [ui_tilt_node_2] -> Abs10/1
  [sigma_bar_w_vec] -> cal differentiator d_sigma_bar_w_hat agent 1/1(x)
  Constant470/1 -> cal Phi_bar_psi_e agent 4/1(pp0)
  [theta_sigma_bar_w_tilt_1_5] -> combine theta_sigma_bar_w_tilt/5(theta_sigma_bar_w_tilt_1_5)
  Mux141/1 -> Interpreted MATLAB Function65/1
  [Si_vec] -> choose ksi_est_err 67/1(x)
  Constant500/1 -> Mux196/2
  Constant487/1 -> cal Fi_S agent 3/1(cS0)
  Constant573/1 -> generate angular rate disturbance agent 5/3(dw_phi_t)
  Mux145/1 -> Interpreted MATLAB Function75/1
  [d2_ui_hat_node_5] -> cal d_theta_hat4/12(d2ui_hat)
  Constant494/1 -> Mux194/2
  cal abs 74/1(y) -> Mux187/1
  [Si_squ_beta_w_1_node_2] -> combine Si_squ_beta_w_1/2(Si_squ_beta_w_1_node_2)
  Mux211/1 -> Interpreted MATLAB Function119/1
  Integrator50/1 -> [sigma_w_5]
  [Si_vec] -> cal theta_Si_beta_w agent 4/4(Si_vec)
  choose ui agent 5/1(y) -> Add19/2
  Constant323/1 -> cal d_theta_hat3/3(c3)
  [Rei_vec] -> cal Fi_S agent 1/7(Rei_vec)
  cal Phi_bar_psi_e agent 1/1(Phi_bar_psi_e_node_1) -> [Phi_bar_psi_e_node_1]
  Constant479/1 -> cal Phi_bar_psi_e agent 5/3(beta_Phi_2)
  [theta_sigma_bar_w_tilt_1_vec] -> cal sigma_bar_w_hat agent 1/3(theta_sigma_bar_w_tilt_1_vec)
  Mux197/1 -> Interpreted MATLAB Function104/1
  [Qci_1] -> cal Rci agent 1/1(Qci)
  [Si_vec] -> cal theta_Si_beta_w agent 3/4(Si_vec)
  Constant621/1 -> Mux158/2
  choose ksi_est_err 66/1(y) -> cal abs 86/1(x)
  [d_sigma_bar_w_vec] -> cal dw_hat agent 2/3(d_sigma_bar_w_vec)
  choose ksi_est_err 65/1(y) -> cal abs 85/1(x)
  [theta_sigma_bar_w_tilt_2_4] -> combine theta_sigma_bar_w_tilt/9(theta_sigma_bar_w_tilt_2_4)
  [Si_squ_beta_w_2_vec] -> cal theta_Si_beta_w agent 3/3(Si_squ_beta_w_2_vec)
  cal sig26/1(z) -> [ui_sig_1_node_5]
  Constant339/1 -> Mux190/2
  [Si_vec] -> choose ksi_est_err 65/1(x)
  [sigma_w_3] -> combine sigma_w/3(sigma_w_3)
  [sigma_bar_w_tilt_vec] -> cal theta_sigma_bar_w_tilt agent 5/4(sigma_bar_w_tilt_vec)
  [Si_vec] -> choose ksi_est_err 62/1(x)
  Constant502/1 -> Mux195/2
  cal theta_Si_beta_w agent 2/2(theta_Si_beta_w_2_node_2) -> [theta_Si_beta_w_2_node_2]
  cal Phi_bar_psi_e agent 4/1(Phi_bar_psi_e_node_4) -> [Phi_bar_psi_e_node_4]
  Constant444/1 -> Mux166/3
  Mux204/1 -> Interpreted MATLAB Function111/1
  Mux168/1 -> Interpreted MATLAB Function92/1
  Constant582/1 -> cal Phi_psi_e agent 3/5(eps_s_bar_div_pi)
  Mux196/1 -> Interpreted MATLAB Function103/1
  [S_bar_node_1] -> combine S_bar/1(S_bar_node_1)
  trans to column99/1(y) -> [V_Phi_Rei_squ_p_min_1_node_4], Display152/1
  Abs12/1 -> Mux145/1
  [Si_squ_beta_w_2_vec] -> cal theta_Si_beta_w agent 2/3(Si_squ_beta_w_2_vec)
  Constant522/1 -> Mux168/3
  Constant508/1 -> Mux197/3
  cal theta_Si_beta_w agent 5/2(theta_Si_beta_w_2_node_5) -> [theta_Si_beta_w_2_node_5]
  Interpreted MATLAB Function66/1 -> trans to column66/1(x)
  Interpreted MATLAB Function65/1 -> trans to column64/1(x)
  Integrator4/1 -> Display126/1, Demux100/1, [d2_ui_hat_node_1]
  [wei_vec] -> cal S_bar agent 2/4(wei_vec)
  [wi_vec] -> cal d_sigma_w agent 3/3(wi_vec)
  cal sigma_bar_w_hat agent 5/1(d_sigma_bar_w_hat_5) -> sigma_bar_w_hat Integrator 5/1
  Constant503/1 -> Mux195/3
  Constant630/1 -> cal d_theta_hat1/3(c3)
  Constant457/1 -> cal dw_hat agent 5/2(Ji)
  [Si_squ_beta_w_1_vec] -> cal theta_Si_beta_w agent 2/2(Si_squ_beta_w_1_vec)
  Demux126/1 -> Mux184/1
  cal abs 81/1(y) -> Mux196/1
  [dwci_vec] -> cal Fi_S agent 2/6(dwci_vec)
  Mux194/1 -> Interpreted MATLAB Function101/1
  Constant506/1 -> Mux209/3
  [wi_vec] -> cal Fi_S agent 4/3(wi_vec)
  Constant497/1 -> Mux193/3
  choose ksi_est_err 75/1(y) -> cal abs 95/1(x)
  cal theta_Si_beta_w agent 1/1(theta_Si_beta_w_1_node_1) -> [theta_Si_beta_w_1_node_1]
  choose ksi_est_err 45/1(y) -> cal abs 65/1(x)
  trans to column101/1(y) -> [Si_squ_beta_w_2_node_1], Display154/1
  [Si_vec] -> cal theta_Si_beta_w agent 5/4(Si_vec)
  [ui_tilt_node_1] -> Abs/1
  choose ui agent 1/1(y) -> Add23/2
  Integrator49/1 -> [sigma_w_4]
  [Qei_4] -> combine wei Qei Rei/9(Qei_4)
  [wei_vec] -> cal S_bar agent 3/4(wei_vec)
  Constant357/1 -> Mux163/2
  cal wei agent 5/1(wei_5) -> [wei_5]
  choose ksi_est_err 52/1(y) -> cal abs 72/1(x)
  cal taui agent 5/1(tau_5) -> [tau_5]
  choose ksi_est_err 64/1(y) -> cal abs 84/1(x)
  [theta_sigma_bar_w_tilt_1_2] -> combine theta_sigma_bar_w_tilt/2(theta_sigma_bar_w_tilt_1_2)
  choose ksi_est_err 60/1(y) -> cal abs 80/1(x)
  Constant629/1 -> Add24/1
  Constant568/1 -> generate angular rate disturbance agent 4/2(dw_ff_t)
  [dw_hat_5] -> combine dw_hat/5(dw_hat_5)
  cal wei agent 2/1(wei_2) -> [wei_2]
  Constant567/1 -> generate angular rate disturbance agent 4/1(dw_aa_t)
  generate angular rate disturbance agent 4/1(dw_4) -> [dw_4]
  Demux139/1 -> d_ui_hat_node_2/1
  cal d_theta_hat2/2(d_dui_hat) -> Integrator8/1
  trans to column75/1(y) -> [ui_squ_6_node_3]
  Abs17/1 -> Mux151/1
  cal abs 80/1(y) -> Mux193/1
  Interpreted MATLAB Function85/1 -> trans to column84/1(x)
  Constant315/1 -> cal d_theta_hat2/4(chi_t)
  [sigma_bar_w_tilt_squ_2_5] -> cal theta_sigma_bar_w_tilt agent 5/3(sigma_bar_w_tilt_squ_2_5)
  Mux151/1 -> Interpreted MATLAB Function74/1
  Constant304/1 -> cal d_theta_hat2/1(c1)
  trans to column74/1(y) -> [ui_squ_4_node_3]
  [ui_squ_4_node_3] -> cal sig12/1(x)
  Integrator8/1 -> Display131/1, Demux129/1, [d_ui_hat_node_3]
  cal wei agent 4/1(wei_4) -> [wei_4]
  cal S_bar agent 3/1(S_bar_node_3) -> [S_bar_node_3]
  Constant310/1 -> Mux150/2
  Product3/1 -> Add26/2
  [ui_tilt_node_2] -> cal sig7/2(y)
  Mux140/1 -> Interpreted MATLAB Function64/1
  Constant371/1 -> Product2/2
  cal abs 82/1(y) -> Mux195/1
  trans to column65/1(y) -> [ui_squ_1_node_2]
  Constant569/1 -> generate angular rate disturbance agent 4/3(dw_phi_t)
  Interpreted MATLAB Function63/1 -> trans to column65/1(x)
  Constant377/1 -> cal S_bar agent 3/1(cS0)
  Mux143/1 -> Interpreted MATLAB Function66/1
  [sigma_bar_w_hat_vec] -> cal combine sigma_bar_w_tilt/2(sigma_bar_w_hat_vec)
  Constant619/1 -> Mux142/2
  [theta_Si_beta_w_2_node_5] -> combine theta_Si_beta_w_2/5(theta_Si_beta_w_2_node_5)
  [wi_2] -> combine dwi/2(wi_2)
  Constant631/1 -> Mux141/3
  [ui_sig_1_node_2] -> cal d_theta_hat1/5(ui_sig_1)
  Demux141/1 -> d_sigma_bar_w_est_5/1
  [d_ui_hat_node_2] -> cal d_theta_hat1/11(dui_hat)
  Integrator6/1 -> Display129/1, Demux101/1, [d2_ui_hat_node_2]
  [ui_tilt_node_2] -> Abs8/1
  [taui_vec] -> wi dynam agent 3/3(taui_vec)
  Product4/1 -> Add29/2
  [ui_sig_6_node_2] -> cal d_theta_hat1/10(ui_sig_6)
  [ui_squ_6_node_2] -> cal sig9/1(x)
  Integrator1/1 -> Display127/1, [ui_hat_node_2]
  [Si_squ_beta_w_2_node_5] -> combine Si_squ_beta_w_2/5(Si_squ_beta_w_2_node_5)
  [ui_tilt_node_2] -> Abs6/1
  combine V_Phi_Rei_squ_2p/1(V_Phi_Rei_squ_2p_vec) -> Memory13/1
  [ui_tilt_node_2] -> cal sig10/2(y)
  Constant305/1 -> cal d_theta_hat2/2(c2)
  Mux146/1 -> Interpreted MATLAB Function70/1
  [V_Phi_Rei_squ_2p_vec] -> cal Phi_bar_psi_e agent 1/12(V_Phi_Rei_squ_2p_vec)
  [wi_vec] -> Qi dynam agent 4/2(wi_vec)
  [dwci_vec] -> cal Fi_S agent 4/6(dwci_vec)
  [V_Phi_Rei_squ_p_plus_1_node_3] -> combine V_Phi_Rei_squ_p_plus_1/3(V_Phi_Rei_squ_p_plus_1_node_3)
  [S_bar_vec] -> cal Phi_psi_e agent 3/6(S_bar_vec)
  trans to column106/1(y) -> [Si_squ_beta_w_2_node_3], Display158/1
  choose ksi_est_err 42/1(y) -> cal abs 62/1(x)
  trans to column125/1(y) -> [ui_squ_6_node_1]
  Constant620/1 -> Mux142/3
  Demux136/1 -> d_sigma_bar_w_est_3/1
  cal Fi_S agent 3/1(Fi_S_3) -> [Fi_S_3]
  cal sig11/1(z) -> [ui_sig_5_node_2]
  [S_bar_node_2] -> combine S_bar/2(S_bar_node_2)
  cal theta_Si_beta_w agent 2/1(theta_Si_beta_w_1_node_2) -> [theta_Si_beta_w_1_node_2]
  Demux116/3 -> wci_node_5/3
  Demux136/3 -> d_sigma_bar_w_est_3/3
  Mux195/1 -> Interpreted MATLAB Function102/1
  trans to column93/1(y) -> [V_Phi_Rei_squ_p_plus_1_node_5], Display122/1
  [S_bar_vec] -> cal Phi_bar_psi_e agent 2/8(S_bar_vec)
  [theta_Si_beta_w_2_node_3] -> combine theta_Si_beta_w_2/3(theta_Si_beta_w_2_node_3)
  [d_ui_hat_node_2] -> combine duihat d2uihat/2(d_ui_hat_node_2)
  [V_Phi_Rei_squ_p_plus_1_vec] -> cal Phi_psi_e agent 4/8(V_Phi_Rei_squ_p_plus_1_vec)
  Constant463/1 -> cal Phi_bar_psi_e agent 3/1(pp0)
  Constant614/1 -> cal Si agent 5/1(cS0)
  [theta_sigma_bar_w_tilt_1_3] -> combine theta_sigma_bar_w_tilt/3(theta_sigma_bar_w_tilt_1_3)
  Interpreted MATLAB Function75/1 -> trans to column75/1(x)
  [dw_hat_vec] -> cal taui agent 5/7(dw_hat_vec)
  cal error dw_tilt/1(dw_tilt_vec) -> [dw_tilt_vec]
  Interpreted MATLAB Function97/1 -> trans to column98/1(x)
  cal abs 79/1(y) -> Mux194/1
  Constant587/1 -> cal Phi_psi_e agent 4/5(eps_s_bar_div_pi)
  [theta_Si_beta_w_1_vec] -> cal taui agent 4/9(theta_Si_beta_w_1_vec)
  Interpreted MATLAB Function89/1 -> trans to column90/1(x)
  [V_Phi_Rei_div_pi_vec] -> cal S_bar agent 3/5(V_Phi_Rei_div_pi_vec)
  Constant407/1 -> Mux200/2
  Constant537/1 -> cal taui agent 4/2(c_w_2)
  Memory24/1 -> [theta_Si_beta_w_2_vec]
  Mux189/1 -> Interpreted MATLAB Function97/1
  trans to column61/1(y) -> [V_Phi_Rei_squ_p_plus_1_node_1], Display96/1
  Mux173/1 -> Scope2/3
  Add12/1 -> Mux145/2
  Constant525/1 -> cal taui agent 1/3(c_w_3)
  Product7/1 -> Add14/2
  [V_Phi_Rei_squ_p_plus_1_vec] -> cal Phi_psi_e agent 5/8(V_Phi_Rei_squ_p_plus_1_vec)
  Constant527/1 -> cal taui agent 2/1(c_w_1)
  [ui_tilt_node_5] -> cal sig26/2(y)
  choose ksi_est_err 74/1(y) -> cal abs 94/1(x)
  [Si_vec] -> cal taui agent 5/6(Si_vec)
  [wi_1] -> combine dwi/1(wi_1)
  Constant542/1 -> cal taui agent 5/3(c_w_3)
  cal d_theta_hat2/1(d_ui_hat) -> Integrator7/1
  Constant396/1 -> cal Phi_bar_psi_e agent 2/2(beta_Phi_1)
  Constant480/1 -> cal Phi_bar_psi_e agent 5/4(thr_p_plus_1)
  choose ksi_est_err 48/1(y) -> cal abs 68/1(x)
  [theta_Si_beta_w_2_vec] -> cal taui agent 5/10(theta_Si_beta_w_2_vec)
  [dw_hat_vec] -> cal taui agent 2/7(dw_hat_vec)
  cal sig9/1(z) -> [ui_sig_6_node_2]
  Constant381/1 -> Product8/2
  Demux126/3 -> Mux183/1
  [Fi_S_1] -> combine Fi_S/1(Fi_S_1)
  combine dw_hat/1(dw_hat_vec) -> [dw_hat_vec]
  Abs16/1 -> Mux150/1
  [V_Phi_Rei_div_pi_vec] -> cal Phi_bar_psi_e agent 1/9(V_Phi_Rei_div_pi_vec)
  Constant538/1 -> cal taui agent 4/3(c_w_3)
  Constant572/1 -> generate angular rate disturbance agent 5/2(dw_ff_t)
  cal Phi_psi_e agent 1/1(Phi_psi_e_node_1) -> [Phi_psi_e_node_1]
  [Phi_bar_psi_e_vec] -> cal Fi_S agent 1/8(Phi_bar_psi_e_vec)
  [S_bar_node_3] -> combine S_bar/3(S_bar_node_3)
  Constant428/1 -> Mux205/3
  [dw_hat_vec] -> cal taui agent 4/7(dw_hat_vec)
  combine wei Qei Rei/1(wei_vec) -> Memory6/1
  [sigma_bar_w_vec] -> cal differentiator d_sigma_bar_w_hat agent 3/1(x)
  Constant499/1 -> Mux167/3
  Interpreted MATLAB Function68/1 -> trans to column68/1(x)
  Constant536/1 -> cal taui agent 4/1(c_w_1)
  cal theta_sigma_bar_w_tilt agent 5/1(theta_sigma_bar_w_tilt_1_5) -> [theta_sigma_bar_w_tilt_1_5]
  cal abs 86/1(y) -> Mux211/1
  [Si_squ_beta_w_2_node_2] -> combine Si_squ_beta_w_2/2(Si_squ_beta_w_2_node_2)
  Mux180/1 -> Interpreted MATLAB Function105/1
  trans to column115/1(y) -> [sigma_bar_w_tilt_squ_1_2], Display102/1
  [V_Phi_Rei_div_pi_vec] -> cal Phi_psi_e agent 5/7(V_Phi_Rei_div_pi_vec)
  Constant402/1 -> Mux199/2
  Interpreted MATLAB Function95/1 -> trans to column96/1(x)
  Constant550/1 -> cal taui agent 1/4(k_J_0)
  Constant368/1 -> Add10/2
  [ui_squ_4_node_4] -> cal sig18/1(x)
  [theta_Si_beta_w_2_vec] -> cal taui agent 3/10(theta_Si_beta_w_2_vec)
  [ui_hat_node_3] -> Add13/1
  Constant553/1 -> cal taui agent 4/4(k_J_0)
  Interpreted MATLAB Function100/1 -> trans to column101/1(x)
  Demux134/1 -> d_sigma_bar_w_est_2/1
  [V_Phi_Rei_squ_p_plus_1_vec] -> cal S_bar agent 1/6(V_Phi_Rei_squ_p_plus_1_vec)
  [theta_Si_beta_w_2_node_4] -> combine theta_Si_beta_w_2/4(theta_Si_beta_w_2_node_4)
  Mux201/1 -> Interpreted MATLAB Function109/1
  Constant551/1 -> cal taui agent 2/4(k_J_0)
  Constant334/1 -> Mux187/3
  [ui_squ_3_node_4] -> cal sig22/1(x)
  [Phi_bar_psi_e_node_2] -> combine Phi_bar_psi_e/2(Phi_bar_psi_e_node_2)
  Constant476/1 -> cal Phi_bar_psi_e agent 5/1(pp0)
  Interpreted MATLAB Function113/1 -> trans to column117/1(x)
  Constant477/1 -> cal S_bar agent 4/3(thr_p_plus_1)
  Constant307/1 -> cal d_theta_hat2/3(c3)
  [V_Phi_Rei_squ_2p_node_5] -> combine V_Phi_Rei_squ_2p/5(V_Phi_Rei_squ_2p_node_5)
  [ui_squ_5_node_3] -> cal sig13/1(x)
  Constant433/1 -> Mux166/2
  [ui_tilt_node_3] -> cal sig17/2(y)
  [wi_vec] -> cal wei agent 1/1(wi_vec)
  [V_Phi_Rei_div_pi_vec] -> choose ksi_est_err 42/1(x)
  Constant464/1 -> cal Phi_bar_psi_e agent 3/2(beta_Phi_1)
  Interpreted MATLAB Function64/1 -> trans to column63/1(x)
  Constant309/1 -> Mux150/3
  cal sig13/1(z) -> [ui_sig_5_node_3]
  Constant539/1 -> cal taui agent 4/5(Ji)
  Constant571/1 -> cal Phi_psi_e agent 1/1(beta_Phi_1)
  [Si_vec] -> cal taui agent 1/6(Si_vec)
  [V_Phi_Rei_div_pi_vec] -> cal Phi_psi_e agent 1/7(V_Phi_Rei_div_pi_vec)
  [Si_squ_beta_w_2_vec] -> cal theta_Si_beta_w agent 4/3(Si_squ_beta_w_2_vec)
  cal theta_Si_beta_w agent 4/2(theta_Si_beta_w_2_node_4) -> [theta_Si_beta_w_2_node_4]
  [ui_sig_3_node_4] -> cal d_theta_hat3/7(ui_sig_3)
  combine Qci Rci/2(Rci_vec) -> Memory17/1
  cal Phi_bar_psi_e agent 3/1(Phi_bar_psi_e_node_3) -> [Phi_bar_psi_e_node_3]
  Constant516/1 -> Mux214/2
  Interpreted MATLAB Function84/1 -> trans to column82/1(x)
  [Fi_S_vec] -> cal taui agent 3/8(Fi_S_vec)
  Abs15/1 -> Mux148/1
  Constant531/1 -> cal taui agent 3/1(c_w_1)
  cal abs 83/1(y) -> Mux158/1
  cal differentiator d_sigma_bar_w_hat agent 5/3(Out3) -> Demux140/1, [d2_sigma_bar_w_est_5], Display168/1
  cal abs 77/1(y) -> Mux190/1
  choose ksi_est_err 67/1(y) -> cal abs 87/1(x)
  Interpreted MATLAB Function119/1 -> trans to column120/1(x)
  [Qei_3] -> combine wei Qei Rei/8(Qei_3)
  [V_Phi_Rei_squ_p_min_1_vec] -> cal Phi_bar_psi_e agent 4/10(V_Phi_Rei_squ_p_min_1_vec)
  Constant300/1 -> Mux169/2
  Demux117/2 -> dwci_node_5/2
  [Si_vec] -> cal taui agent 3/6(Si_vec)
  Constant450/1 -> cal dw_hat agent 3/2(Ji)
  Interpreted MATLAB Function91/1 -> trans to column91/1(x)
  [Rci_4] -> combine Qci Rci/9(Rci_4)
  Constant442/1 -> cal sigma_bar_w_hat agent 5/1(h1w)
  [Phi_psi_e_vec] -> cal Si agent 4/3(Phi_psi_e_vec)
  [sigma_w_vec] -> cal sigma_w_bar/2(sigma_w_vec)
  [wei_2] -> combine wei Qei Rei/2(wei_2)
  Add27/1 -> Demux110/1, [ui_tilt_node_2]
  [theta_Si_beta_w_1_vec] -> cal taui agent 3/9(theta_Si_beta_w_1_vec)
  Product5/1 -> Add12/2
  Constant394/1 -> cal Phi_bar_psi_e agent 1/6(eps_s_bar_div_pi)
  Memory12/1 -> [V_Phi_Rei_vec]
  cal abs 85/1(y) -> Mux197/1
  [ui_sig_4_node_5] -> cal d_theta_hat4/8(ui_sig_4)
  Integrator24/1 -> [wi_4]
  cal S_bar agent 4/1(S_bar_node_4) -> [S_bar_node_4]
  [Rei_vec] -> cal wei agent 2/2(Rei_vec)
  trans to column112/1(y) -> [sigma_bar_w_tilt_squ_2_4], Display106/1
  [Phi_psi_e_vec] -> cal Si agent 1/3(Phi_psi_e_vec)
  Constant299/1 -> Mux136/2
  [sigma_bar_w_tilt_vec] -> choose ksi_est_err 51/1(x)
  Constant608/1 -> cal Phi_psi_e agent 5/1(beta_Phi_1)
  Abs6/1 -> Mux142/1
  [Si_vec] -> cal taui agent 4/6(Si_vec)
  cal sig19/1(z) -> [ui_sig_5_node_4]
  [theta_Si_beta_w_2_node_2] -> combine theta_Si_beta_w_2/2(theta_Si_beta_w_2_node_2)
  cal wci dwci agent 5/1(wci) -> Display150/1, Demux116/1, [wci_node_5]
  [Fi_S_2] -> combine Fi_S/2(Fi_S_2)
  [tau_3] -> combine tau/3(tau_3)
  [Rei_vec] -> cal Fi_S agent 3/7(Rei_vec)
  Constant460/1 -> cal d_sigma_w agent 5/1(h3w)
  Constant372/1 -> Product3/2
  trans to column97/1(y) -> [V_Phi_Rei_squ_p_min_1_node_2], Display140/1
  [ui_squ_2_node_4] -> cal sig21/1(x)
  trans to column80/1(y) -> [ui_squ_4_node_4]
  Integrator42/1 -> [V_Phi_Rei_4]
  Integrator32/1 -> [Qei_2]
  Constant554/1 -> cal taui agent 5/4(k_J_0)
  cal theta_sigma_bar_w_tilt agent 5/2(theta_sigma_bar_w_tilt_2_5) -> [theta_sigma_bar_w_tilt_2_5]
  Constant532/1 -> cal taui agent 3/2(c_w_2)
  Constant455/1 -> cal S_bar agent 4/1(cS0)
  [Qi_1] -> combine Qi Ri/1(Qi_1)
  Memory18/1 -> [Phi_psi_e_vec]
  [theta_Si_beta_w_1_vec] -> cal taui agent 2/9(theta_Si_beta_w_1_vec)
  Interpreted MATLAB Function124/1 -> trans to column125/1(x)
  Constant417/1 -> Mux204/2
  Mux169/1 -> Interpreted MATLAB Function94/1
  [S_bar_vec] -> cal Phi_psi_e agent 5/6(S_bar_vec)
  [ui_sig_1_node_3] -> cal d_theta_hat2/5(ui_sig_1)
  [ui_tilt_node_3] -> cal sig15/2(y)
  cal theta_sigma_bar_w_tilt agent 4/1(theta_sigma_bar_w_tilt_1_4) -> [theta_sigma_bar_w_tilt_1_4]
  cal wci dwci agent 3/2(dwci) -> [dwci_node_3], Display147/1, Demux113/1
  Constant312/1 -> Mux151/3
  Mux214/1 -> Interpreted MATLAB Function121/1
  Interpreted MATLAB Function94/1 -> trans to column94/1(x)
  Demux109/3 -> dwci_node_2/3
  [sigma_bar_w_tilt_vec] -> choose ksi_est_err 49/1(x)
  Constant592/1 -> Add22/1
  [ui_squ_1_node_4] -> cal sig20/1(x)
  Demux107/1 -> wci_node_2/1
  Constant298/1 -> Mux202/2
  combine theta_Si_beta_w_2/1(theta_Si_beta_w_2_vec) -> Memory24/1
  Demux114/2 -> wci_node_4/2
  [ui_vec] -> choose ui agent 2/1(x)
  [theta_sigma_bar_w_tilt_2_3] -> combine theta_sigma_bar_w_tilt/8(theta_sigma_bar_w_tilt_2_3)
  Mux142/1 -> Interpreted MATLAB Function63/1
  Constant344/1 -> cal S_bar agent 2/3(thr_p_plus_1)
  Demux112/2 -> wci_node_3/2
  [d_ui_hat_node_3] -> combine duihat d2uihat/3(d_ui_hat_node_3)
  [wci_vec] -> cal Fi_S agent 3/4(wci_vec)
  [Fi_S_3] -> combine Fi_S/3(Fi_S_3)
  Interpreted MATLAB Function71/1 -> trans to column70/1(x)
  [ui_squ_5_node_1] -> cal sig5/1(x)
  choose ksi_est_err 68/1(y) -> cal abs 88/1(x)
  [ui_tilt_node_4] -> Abs18/1
  [Si_squ_beta_w_1_vec] -> cal theta_Si_beta_w agent 3/2(Si_squ_beta_w_1_vec)
  Demux100/3 -> d2_ui_hat_node_1/3
  trans to column110/1(y) -> [sigma_bar_w_tilt_squ_2_3], Display103/1
  Demux104/3 -> d2_ui_hat_node_5/3
  [dwci_vec] -> cal Fi_S agent 5/6(dwci_vec)
  Demux106/1 -> dwci_node_1/1
  [dwci_vec] -> cal Fi_S agent 1/6(dwci_vec)
  [sigma_w_2] -> combine sigma_w/2(sigma_w_2)
  [ui_squ_6_node_3] -> cal sig17/1(x)
  Constant342/1 -> Mux192/3
  Demux111/2 -> ui_tilt_node_3/2
  [Rei_vec] -> cal Fi_S agent 4/7(Rei_vec)
  [taui_vec] -> cal d_sigma_w agent 5/4(taui_vec)
  Constant507/1 -> Mux197/2
  Demux110/3 -> ui_tilt_node_2/3
  Constant401/1 -> cal d_sigma_w agent 5/2(Ji)
  Demux111/1 -> ui_tilt_node_3/1
  [Rei_3] -> combine wei Qei Rei/13(Rei_3)
  Demux139/3 -> d_ui_hat_node_2/3
  Demux129/3 -> d_ui_hat_node_3/3
  Demux128/2 -> ui_tilt_node_5/2
  [Ri_2] -> combine Qi Ri/7(Ri_2)
  cal wci dwci agent 5/2(dwci) -> Display151/1, Demux117/1, [dwci_node_5]
  [sigma_bar_w_tilt_vec] -> choose ksi_est_err 47/1(x)
  cal d_theta_hat1/3(d_d2ui_hat) -> Integrator6/1
  Abs19/1 -> Mux153/1
  Mux210/1 -> Interpreted MATLAB Function118/1
  [wci_node_4] -> combine wci dwci/4(wci_node_4)
  [Rci_vec] -> cal wci dwci agent 5/4(Rci_mat)
  [wci_node_2] -> combine wci dwci/2(wci_node_2)
  [ui_tilt_node_5] -> cal sig27/2(y)
  Constant325/1 -> Mux156/3
  [sigma_bar_w_tilt_squ_2_4] -> cal theta_sigma_bar_w_tilt agent 4/3(sigma_bar_w_tilt_squ_2_4)
  Constant400/1 -> cal d_sigma_w agent 1/1(h3w)
  [ui_vec] -> cal wci dwci agent 5/1(ui_vec)
  trans to column73/1(y) -> [ui_squ_3_node_3]
  Constant505/1 -> Mux209/2
  Mux170/1 -> Interpreted MATLAB Function93/1
  [ui_tilt_node_3] -> Abs14/1
  [wci_vec] -> cal wei agent 4/3(wci_vec)
  Integrator5/1 -> Display128/1, [d_ui_hat_node_2], Demux139/1
  [Si_squ_beta_w_1_vec] -> cal theta_Si_beta_w agent 5/2(Si_squ_beta_w_1_vec)
  [taui_vec] -> wi dynam agent 4/3(taui_vec)
  trans to column96/1(y) -> [V_Phi_Rei_squ_p_min_1_node_1], Display139/1
  [wei_4] -> Integrator42/1
  [V_Phi_Rei_squ_2p_node_4] -> combine V_Phi_Rei_squ_2p/4(V_Phi_Rei_squ_2p_node_4)
  [wei_1] -> Integrator20/1
  Memory22/1 -> [Si_squ_beta_w_2_vec]
  Abs24/1 -> Mux159/1
  Constant437/1 -> cal d_sigma_w agent 2/2(Ji)
  Mux158/1 -> Interpreted MATLAB Function83/1
  Demux124/1 -> Mux181/1
  Constant640/1 -> Mux149/3
  [Qci_2] -> cal Rci agent 2/1(Qci)
  [ui_tilt_node_1] -> Abs5/1
  Memory17/1 -> [Rci_vec]
  Constant543/1 -> cal taui agent 5/5(Ji)
  cal d_theta_hat/3(d_d2ui_hat) -> Integrator4/1
  cal abs 88/1(y) -> Mux214/1
  Memory15/1 -> Display101/1, [dwci_vec]
  [Qci_3] -> cal Rci agent 3/1(Qci)
  Demux114/3 -> wci_node_4/3
  Constant637/1 -> Product2/1
  Constant462/1 -> cal Phi_bar_psi_e agent 2/6(eps_s_bar_div_pi)
  [ui_tilt_node_2] -> cal sig9/2(y)
  cal Rci agent 1/1(Rci_1) -> [Rci_1]
  cal theta_Si_beta_w agent 4/1(theta_Si_beta_w_1_node_4) -> [theta_Si_beta_w_1_node_4]
  Constant385/1 -> wi dynam agent 3/1(Ji)
  Constant534/1 -> cal taui agent 3/3(c_w_3)
  Add28/1 -> Mux148/2
  Constant552/1 -> cal taui agent 3/4(k_J_0)
  Memory16/1 -> [Qci_vec]
  Mux215/1 -> Interpreted MATLAB Function123/1
  [ui_vec] -> cal wci dwci agent 2/1(ui_vec)
  Demux133/3 -> d2_sigma_bar_w_est_2/3
  cal Rci agent 5/1(Rci_5) -> [Rci_5]
  Constant332/1 -> Mux187/2
  cal Fi_S agent 4/1(Fi_S_4) -> [Fi_S_4]
  cal Qci agent 2/1(Qci_2) -> [Qci_2]
  Demux108/2 -> ui_tilt_node_1/2
  [ui_vec] -> choose ui agent 3/1(x)
  cal differentiator d_sigma_bar_w_hat agent 3/1(Out1) -> Display114/1, [sigma_bar_w_est_3]
  trans to column68/1(y) -> [ui_squ_6_node_2]
  Interpreted MATLAB Function67/1 -> trans to column67/1(x)
  Memory5/1 -> [wi_vec]
  [sigma_bar_w_hat_4] -> combine sigma_bar_w_hat/4(sigma_bar_w_hat_4)
  Constant598/1 -> Add10/1
  choose ksi_est_err 47/1(y) -> cal abs 67/1(x)
  [Si_squ_beta_w_2_vec] -> cal theta_Si_beta_w agent 1/3(Si_squ_beta_w_2_vec)
  Constant367/1 -> Add24/2
  choose ksi_est_err 61/1(y) -> cal abs 81/1(x)
  cal sig25/1(z) -> [ui_sig_5_node_5]
  cal Rci agent 2/1(Rci_2) -> [Rci_2]
  Demux105/1 -> wci_node_1/1
  Interpreted MATLAB Function121/1 -> trans to column122/1(x)
  Add23/1 -> Demux108/1, [ui_tilt_node_1]
  Demux101/2 -> d2_ui_hat_node_2/2
  [wi_vec] -> wi dynam agent 5/2(wi_vec)
  [d_sigma_bar_w_est_4] -> combine d_sigma_bar_v_est1/4(d_sigma_bar_w_est_4)
  [ui_tilt_node_3] -> Abs12/1
  Constant642/1 -> Add12/1
  [d_sigma_bar_w_est_1] -> combine d_sigma_bar_v_est1/1(d_sigma_bar_w_est_1)
  [Si_5] -> combine Si/5(Si_5)
  [ui_tilt_node_2] -> cal sig8/2(y)
  [wci_vec] -> cal wei agent 2/3(wci_vec)
  [ui_hat_node_5] -> Demux126/1
  [Qi_vec] -> cal Qci agent 5/1(Qi_vec)
  Mux154/1 -> Interpreted MATLAB Function78/1
  [Si_squ_beta_w_1_vec] -> cal theta_Si_beta_w agent 4/2(Si_squ_beta_w_1_vec)
  Demux/1 -> Mux171/1
  trans to column70/1(y) -> [ui_squ_2_node_3]
  Demux113/1 -> dwci_node_3/1
  combine theta_Si_beta_w_1/1(theta_Si_beta_w_1_vec) -> Memory23/1
  [ui_hat_node_2] -> Add27/1
  Constant432/1 -> cal sigma_bar_w_hat agent 1/1(h1w)
  [Qei_vec] -> Qei dynam agent 5/1(Qei_vec)
  cal d_theta_hat1/2(d_dui_hat) -> Integrator5/1
  Add16/1 -> Mux154/2
  [V_Phi_Rei_2] -> combine Qci Rci1/2(V_Phi_Rei_2)
  [Si_vec] -> choose ksi_est_err 60/1(x)
  [Rci_3] -> combine Qci Rci/8(Rci_3)
  [Si_vec] -> choose ksi_est_err 64/1(x)
  Constant541/1 -> cal taui agent 5/2(c_w_2)
  Integrator17/1 -> [V_Phi_Rei_2]
  [ui_tilt_node_1] -> Abs4/1
  generate angular rate disturbance agent 1/1(dw_1) -> [dw_1]
  [theta_Si_beta_w_1_node_1] -> combine theta_Si_beta_w_1/1(theta_Si_beta_w_1_node_1)
  Integrator20/1 -> [V_Phi_Rei_1]
  Mux213/1 -> Interpreted MATLAB Function122/1
  trans to column123/1(y) -> [ui_squ_3_node_1]
  Interpreted MATLAB Function118/1 -> trans to column119/1(x)
  [Qi_vec] -> cal Qci agent 3/1(Qi_vec)
  [Qi_vec] -> cal Qci agent 2/1(Qi_vec)
  [Si_squ_beta_w_2_node_4] -> combine Si_squ_beta_w_2/4(Si_squ_beta_w_2_node_4)
  [ui_sig_3_node_1] -> cal d_theta_hat/7(ui_sig_3)
  cal d_theta_hat2/3(d_d2ui_hat) -> Integrator9/1
  Demux114/1 -> wci_node_4/1
  [Qci_4] -> combine Qci Rci/4(Qci_4)
  [Qei_vec] -> cal Qci agent 2/2(Qei_vec)
  [Qei_vec] -> cal Qci agent 5/2(Qei_vec)
  [V_Phi_Rei_div_pi_vec] -> choose ksi_est_err 63/1(x)
  trans to column117/1(y) -> [sigma_bar_w_tilt_squ_1_5], Display112/1
  cal Rci agent 3/1(Rci_3) -> [Rci_3]
  cal sig23/1(z) -> [ui_sig_6_node_4]
  Constant518/1 -> Mux212/2
  [Ri_4] -> combine Qi Ri/9(Ri_4)
  [sigma_bar_w_tilt_squ_1_1] -> cal theta_sigma_bar_w_tilt agent 1/2(sigma_bar_w_tilt_squ_1_1)
  Demux138/3 -> d_sigma_bar_w_est_4/3
  Interpreted MATLAB Function101/1 -> trans to column102/1(x)
  [Ri_5] -> combine Qi Ri/10(Ri_5)
  Demux120/2 -> ui_tilt_node_4/2
  Interpreted MATLAB Function109/1 -> trans to column111/1(x)
  Demux118/2 -> Mux172/2
  [Qi_vec] -> cal Qci agent 1/1(Qi_vec)
  [V_Phi_Rei_squ_2p_node_1] -> combine V_Phi_Rei_squ_2p/1(V_Phi_Rei_squ_2p_node_1)
  [Ri_3] -> combine Qi Ri/8(Ri_3)
  Constant577/1 -> Mux147/3
  [Si_vec] -> choose ksi_est_err 59/1(x)
  Demux121/3 -> Mux174/2
  [d2_ui_hat_node_3] -> combine duihat d2uihat/8(d2_ui_hat_node_3)
  trans to column63/1(y) -> [ui_squ_5_node_2]
  Demux98/2 -> d_ui_hat_node_4/2
  cal differentiator d_sigma_bar_w_hat agent 4/2(Out2) -> Demux138/1, [d_sigma_bar_w_est_4], Display165/1
  [Qi_vec] -> cal Ri agent 4/1(Qi_vec)
  [Qei_5] -> combine wei Qei Rei/10(Qei_5)
  cal taui agent 4/1(tau_4) -> [tau_4]
  [ui_vec] -> cal wci dwci agent 4/1(ui_vec)
  Demux108/1 -> ui_tilt_node_1/1
  Demux109/2 -> dwci_node_2/2
  combine wei Qei Rei/3(Rei_vec) -> Memory8/1
  Constant346/1 -> Add14/1
  [dw_hat_1] -> combine dw_hat/1(dw_hat_1)
  trans to column92/1(y) -> [V_Phi_Rei_squ_2p_node_4], Display121/1
  [Qi_vec] -> cal Ri agent 2/1(Qi_vec)
  Demux130/1 -> d_ui_hat_node_1/1
  [wci_vec] -> cal wei agent 5/3(wci_vec)
  [ui_sig_2_node_2] -> cal d_theta_hat1/6(ui_sig_2)
  [ui_tilt_node_4] -> cal sig18/2(y)
  cal Rei agent 4/1(Rei_4) -> [Rei_4]
  Integrator34/1 -> [Qei_4]
  [wei_3] -> combine wei Qei Rei/3(wei_3)
  Interpreted MATLAB Function83/1 -> trans to column83/1(x)
  Constant471/1 -> cal Phi_bar_psi_e agent 4/2(beta_Phi_1)
  [tau_4] -> combine tau/4(tau_4)
  [wei_vec] -> Qei dynam agent 4/2(wei_vec)
  Demux107/3 -> wci_node_2/3
  Constant361/1 -> cal d_theta_hat4/4(chi_t)
  trans to column102/1(y) -> [Si_squ_beta_w_1_node_1], Display155/1
  [Qei_vec] -> cal Rei agent 3/1(Qei_vec)
  sigma_bar_w_hat Integrator 5/1 -> [sigma_bar_w_hat_5]
  trans to column113/1(y) -> [sigma_bar_w_tilt_squ_1_4], Display109/1
  [Rei_vec] -> cal wei agent 1/2(Rei_vec)
  Mux150/1 -> Interpreted MATLAB Function73/1
  [sigma_bar_w_hat_3] -> combine sigma_bar_w_hat/3(sigma_bar_w_hat_3)
  choose ksi_est_err 63/1(y) -> cal abs 83/1(x)
  Qei dynam agent 1/1(dQei_1) -> Integrator31/1
  Constant634/1 -> Mux143/2
  [V_Phi_Rei_1] -> combine Qci Rci1/1(V_Phi_Rei_1)
  [wei_vec] -> Qei dynam agent 1/2(wei_vec)
  Demux99/3 -> d_ui_hat_node_5/3
  Qei dynam agent 2/1(dQei_2) -> Integrator32/1
  Demux102/1 -> d2_ui_hat_node_3/1
  [wci_vec] -> cal wei agent 1/3(wci_vec)
  [ui_tilt_node_1] -> cal sig3/2(y)
  cal abs 94/1(y) -> Mux166/1
  [Qei_vec] -> cal Rei agent 1/1(Qei_vec)
  Constant636/1 -> Add25/1
  [theta_Si_beta_w_1_node_3] -> combine theta_Si_beta_w_1/3(theta_Si_beta_w_1_node_3)
  [Qi_2] -> combine Qi Ri/2(Qi_2)
  [Qi_5] -> combine Qi Ri/5(Qi_5)
  Constant623/1 -> Add26/1
  Demux103/3 -> d2_ui_hat_node_4/3
  Integrator19/1 -> [V_Phi_Rei_3]
  Constant320/1 -> cal d_theta_hat3/2(c2)
  cal sig22/1(z) -> [ui_sig_3_node_4]
  [Qi_vec] -> Qi dynam agent 3/1(Qi_vec)
  Constant461/1 -> cal Phi_bar_psi_e agent 2/5(gamma0)
  [wi_vec] -> Qi dynam agent 5/2(wi_vec)
  [Qi_vec] -> cal Ri agent 1/1(Qi_vec)
  [wi_vec] -> Qi dynam agent 1/2(wi_vec)
  [Si_3] -> combine Si/3(Si_3)
  [Si_vec] -> choose ksi_est_err 69/1(x)
  Integrator30/1 -> [Qi_5]
  Constant328/1 -> Add17/1
  [sigma_bar_w_tilt_squ_1_2] -> cal theta_sigma_bar_w_tilt agent 2/2(sigma_bar_w_tilt_squ_1_2)
  choose ksi_est_err 44/1(y) -> cal abs 64/1(x)
  Integrator26/1 -> [Qi_1]
  Qi dynam agent 5/1(dQi_5) -> Integrator30/1
  [ui_tilt_node_3] -> Abs17/1
  Demux106/3 -> dwci_node_1/3
  [V_Phi_Rei_squ_p_min_1_vec] -> cal Phi_bar_psi_e agent 1/10(V_Phi_Rei_squ_p_min_1_vec)
  Mux137/1 -> Interpreted MATLAB Function124/1
  Constant387/1 -> wi dynam agent 5/1(Ji)
  Integrator23/1 -> [wi_3]
  Constant504/1 -> cal theta_Si_beta_w agent 2/1(mu_c_theta)
  [V_Phi_Rei_vec] -> cal divide pi/1(x)
  Integrator22/1 -> [wi_2]
  cal theta_sigma_bar_w_tilt agent 4/2(theta_sigma_bar_w_tilt_2_4) -> [theta_sigma_bar_w_tilt_2_4]
  Demux120/1 -> ui_tilt_node_4/1
  [wei_1] -> combine wei Qei Rei/1(wei_1)
  [sigma_bar_w_tilt_vec] -> choose ksi_est_err 46/1(x)
  [sigma_bar_w_tilt_vec] -> cal theta_sigma_bar_w_tilt agent 4/4(sigma_bar_w_tilt_vec)
  Constant556/1 -> Mux170/2
  trans to column62/1(y) -> [ui_squ_5_node_1]
  combine dwi/1(wi_vec) -> Memory5/1
  trans to column64/1(y) -> [ui_squ_2_node_2]
  [Si_vec] -> choose ksi_est_err 68/1(x)
  [taui_vec] -> wi dynam agent 5/3(taui_vec)
  Constant302/1 -> Mux146/3
  [d2_ui_hat_node_1] -> cal d_theta_hat/12(d2ui_hat)
  [Rei_2] -> combine wei Qei Rei/12(Rei_2)
  Integrator25/1 -> [wi_5]
  [ui_tilt_node_1] -> cal sig1/2(y)
  cal sig12/1(z) -> [ui_sig_4_node_3]
  Integrator21/1 -> [wi_1]
  Constant519/1 -> Mux212/3
  [wi_5] -> combine dwi/5(wi_5)
  [d2uihat_vec] -> cal wci dwci agent 5/3(d2uihat_vec)
  [wei_vec] -> cal Phi_bar_psi_e agent 2/7(wei_vec)
  Constant578/1 -> cal Phi_psi_e agent 2/3(gamma0)
  [taui_vec] -> wi dynam agent 2/3(taui_vec)
  Constant624/1 -> Product3/1
  [Qei_2] -> combine wei Qei Rei/7(Qei_2)
  [V_Phi_Rei_squ_p_min_1_vec] -> cal Phi_bar_psi_e agent 5/10(V_Phi_Rei_squ_p_min_1_vec)
  [tau_2] -> combine tau/2(tau_2)
  Constant384/1 -> wi dynam agent 2/1(Ji)
  wi dynam agent 2/1(dwi_2) -> Integrator22/1
  [Phi_bar_psi_e_node_5] -> combine Phi_bar_psi_e/5(Phi_bar_psi_e_node_5)
  [Rei_vec] -> cal wei agent 4/2(Rei_vec)
  Demux98/1 -> d_ui_hat_node_4/1
  Constant375/1 -> Product5/2
  [Qci_1] -> combine Qci Rci/1(Qci_1)
  [Phi_psi_e_vec] -> cal Si agent 3/3(Phi_psi_e_vec)
  Demux127/3 -> Mux183/2
  [ui_n_2] -> Demux121/1
  Constant451/1 -> cal d_sigma_w agent 3/2(Ji)
  Mux174/1 -> Scope1/3
  Constant615/1 -> Mux215/3
  [theta_Si_beta_w_2_node_1] -> combine theta_Si_beta_w_2/1(theta_Si_beta_w_2_node_1)
  Demux113/2 -> dwci_node_3/2
  Integrator46/1 -> [sigma_w_1]
  combine Qci Rci/1(Qci_vec) -> Memory16/1
  trans to column109/1(y) -> [sigma_bar_w_tilt_squ_2_2], Display172/1
  Demux119/3 -> Mux174/1
  [ui_hat_node_1] -> Demux/1
  combine Si/1(Si_vec) -> Memory19/1
  Demux123/3 -> Mux175/2
  [ui_sig_3_node_3] -> cal d_theta_hat2/7(ui_sig_3)
  [duihat_vec] -> cal wci dwci agent 4/2(duihat_vec)
  [ui_n_4] -> Demux125/1
  Demux110/1 -> ui_tilt_node_2/1
  Constant330/1 -> cal d_theta_hat3/4(chi_t)
  [ui_squ_6_node_4] -> cal sig23/1(x)
  [ui_n_5] -> Demux127/1
  [V_Phi_Rei_5] -> combine Qci Rci1/5(V_Phi_Rei_5)
  [ui_tilt_node_3] -> cal sig12/2(y)
  Demux123/1 -> Mux176/2
  Constant340/1 -> Mux190/3
  [Si_squ_beta_w_1_node_3] -> combine Si_squ_beta_w_1/3(Si_squ_beta_w_1_node_3)
  [Rci_1] -> combine Qci Rci/6(Rci_1)
  [Qci_4] -> cal Rci agent 4/1(Qci)
  [ui_hat_node_1] -> Add23/1
  [ui_n_3] -> Demux123/1
  [Rei_1] -> combine wei Qei Rei/11(Rei_1)
  Constant374/1 -> Product4/2
  [ui_tilt_node_1] -> cal sig2/2(y)
  Add17/1 -> Mux157/2
  Constant425/1 -> cal d_sigma_w agent 2/1(h3w)
  cal wei agent 1/1(wei_1) -> [wei_1]
  [Qei_vec] -> cal Qci agent 1/2(Qei_vec)
  Mux184/1 -> Scope15/1
  Constant390/1 -> cal Phi_bar_psi_e agent 1/2(beta_Phi_1)
  [d2uihat_vec] -> cal wci dwci agent 3/3(d2uihat_vec)
  Constant513/1 -> Mux210/2
  Demux117/1 -> dwci_node_5/1
  cal theta_Si_beta_w agent 5/1(theta_Si_beta_w_1_node_5) -> [theta_Si_beta_w_1_node_5]
  Mux193/1 -> Interpreted MATLAB Function100/1
  combine wci dwci/2(dwci_vec) -> Memory15/1
  Integrator35/1 -> [Qei_5]
  Demux126/2 -> Mux185/1
  trans to column86/1(y) -> [ui_squ_3_node_5]
  Demux105/3 -> wci_node_1/3
  [Fi_S_vec] -> cal taui agent 4/8(Fi_S_vec)
  choose ksi_est_err 72/1(y) -> cal abs 92/1(x)
  [wi_vec] -> cal wei agent 5/1(wi_vec)
  [theta_sigma_bar_w_tilt_2_1] -> combine theta_sigma_bar_w_tilt/6(theta_sigma_bar_w_tilt_2_1)
  Demux121/1 -> Mux178/2
  [V_Phi_Rei_squ_p_min_1_vec] -> cal Phi_bar_psi_e agent 2/10(V_Phi_Rei_squ_p_min_1_vec)
  combine wci dwci/1(wci_vec) -> Memory14/1
  Add14/1 -> Mux152/2
  cal Qci agent 3/1(Qci_3) -> [Qci_3]
  Interpreted MATLAB Function114/1 -> trans to column115/1(x)
  cal Qci agent 1/1(Qci_1) -> [Qci_1]
  Constant607/1 -> cal Phi_psi_e agent 5/3(gamma0)
  [ui_hat_node_4] -> Demux124/1
  Demux98/3 -> d_ui_hat_node_4/3
  Mux152/1 -> Interpreted MATLAB Function81/1
  Demux115/2 -> dwci_node_4/2
  Constant350/1 -> cal d_theta_hat4/1(c1)
  Add26/1 -> Mux139/2
  Constant354/1 -> Mux161/3
  [Qei_vec] -> Qei dynam agent 4/1(Qei_vec)
  [Fi_S_vec] -> cal taui agent 2/8(Fi_S_vec)
  Interpreted MATLAB Function120/1 -> trans to column121/1(x)
  [wci_node_3] -> combine wci dwci/3(wci_node_3)
  Constant510/1 -> Mux168/2
  Demux118/3 -> Mux173/2
  Constant566/1 -> generate angular rate disturbance agent 3/3(dw_phi_t)
  Demux122/1 -> Mux176/1
  Constant589/1 -> cal Phi_psi_e agent 4/3(gamma0)
  Constant523/1 -> cal taui agent 1/1(c_w_1)
  Constant565/1 -> generate angular rate disturbance agent 3/2(dw_ff_t)
  generate angular rate disturbance agent 3/1(dw_3) -> [dw_3]
  cal dw_hat agent 4/1(dw_hat_4) -> [dw_hat_4]
  [wi_vec] -> wi dynam agent 4/2(wi_vec)
  Integrator33/1 -> [Qei_3]
  [tsim] -> generate angular rate disturbance agent 3/4(t)
  Constant535/1 -> cal taui agent 3/5(Ji)
  Constant459/1 -> cal d_sigma_w agent 4/2(Ji)
  Mux183/1 -> Scope15/3
  [d2_ui_hat_node_2] -> cal d_theta_hat1/12(d2ui_hat)
  cal sig29/1(z) -> [ui_sig_6_node_5]
  [Qei_vec] -> cal Rei agent 4/1(Qei_vec)
  cal sigma_w_bar/1(sigma_bar_w_vec) -> [sigma_bar_w_vec]
  [ui_sig_1_node_5] -> cal d_theta_hat4/5(ui_sig_1)
  Add20/1 -> Mux161/2
  cal Qci agent 5/1(Qci_5) -> [Qci_5]
  cal d_theta_hat3/3(d_d2ui_hat) -> Integrator12/1
  Product9/1 -> Add18/2
  [ui_tilt_node_4] -> Abs22/1
  Constant597/1 -> cal d_theta_hat/2(c2)
  Constant580/1 -> cal Phi_psi_e agent 2/2(beta_Phi_2)
  [sigma_bar_w_tilt_vec] -> choose ksi_est_err 48/1(x)
  Mux162/1 -> Interpreted MATLAB Function82/1
  [wi_vec] -> wi dynam agent 1/2(wi_vec)
  cal abs 90/1(y) -> Mux169/1
  [ui_tilt_node_3] -> cal sig14/2(y)
  [ui_tilt_node_5] -> Abs27/1
  Constant562/1 -> generate angular rate disturbance agent 2/2(dw_ff_t)
  combine Qi Ri/1(Qi_vec) -> Memory3/1
  [wi_vec] -> cal Fi_S agent 2/3(wi_vec)
  [d_ui_hat_node_5] -> cal d_theta_hat4/11(dui_hat)
  Constant447/1 -> cal dw_hat agent 2/2(Ji)
  cal sig28/1(z) -> [ui_sig_3_node_5]
  Constant509/1 -> cal theta_Si_beta_w agent 3/1(mu_c_theta)
  Constant383/1 -> wi dynam agent 1/1(Ji)
  [ui_tilt_node_3] -> cal sig16/2(y)
  Mux185/1 -> Scope15/2
  [V_Phi_Rei_div_pi_vec] -> choose ksi_est_err 52/1(x)
  Mux199/1 -> Interpreted MATLAB Function107/1
  [ui_squ_3_node_5] -> cal sig28/1(x)
  Interpreted MATLAB Function69/1 -> trans to column71/1(x)
  Mux160/1 -> Interpreted MATLAB Function84/1
  Interpreted MATLAB Function73/1 -> trans to column73/1(x)
  Demux124/2 -> Mux182/1
  [ui_sig_3_node_5] -> cal d_theta_hat4/7(ui_sig_3)
  Integrator44/1 -> [V_Phi_Rei_5]
  Constant362/1 -> Mux162/2
  cal S_bar agent 5/1(S_bar_node_5) -> [S_bar_node_5]
  Constant349/1 -> Mux160/2
  [V_Phi_Rei_div_pi_vec] -> choose ksi_est_err 57/1(x)
  Constant498/1 -> cal theta_Si_beta_w agent 1/1(mu_c_theta)
  Constant352/1 -> Add20/1
  [ui_tilt_node_5] -> Abs28/1
  cal d_theta_hat3/1(d_ui_hat) -> Integrator10/1
  [dwci_node_2] -> combine wci dwci/7(dwci_node_2)
  trans to column103/1(y) -> [Si_squ_beta_w_2_node_2], Display156/1
  trans to column87/1(y) -> [ui_squ_4_node_5]
  Abs25/1 -> Mux160/1
  [Qci_3] -> combine Qci Rci/3(Qci_3)
  cal Si agent 2/1(Si_2) -> [Si_2]
  trans to column78/1(y) -> [ui_squ_1_node_4]
  cal sig14/1(z) -> [ui_sig_1_node_3]
  [wei_vec] -> cal Phi_bar_psi_e agent 1/7(wei_vec)
  [ui_sig_4_node_2] -> cal d_theta_hat1/8(ui_sig_4)
  [sigma_bar_w_vec] -> cal d_sigma_w agent 5/5(sigma_w_bar_vec)
  combine theta_sigma_bar_w_tilt/1(theta_sigma_bar_w_tilt_1_vec) -> [theta_sigma_bar_w_tilt_1_vec]
  Demux122/2 -> Mux177/1
  Product8/1 -> Add21/2
  cal Phi_psi_e agent 4/1(Phi_psi_e_node_4) -> [Phi_psi_e_node_4]
  Demux112/1 -> wci_node_3/1
  [ui_squ_2_node_5] -> cal sig27/1(x)
  Interpreted MATLAB Function88/1 -> trans to column88/1(x)
  Abs29/1 -> Mux164/1
  Constant530/1 -> cal taui agent 2/5(Ji)
  Constant409/1 -> Mux201/2
  choose ksi_est_err 59/1(y) -> cal abs 79/1(x)
  Add15/1 -> Demux120/1, [ui_tilt_node_4]
  Demux119/2 -> Mux186/1
  [Qi_vec] -> Qi dynam agent 4/1(Qi_vec)
  [dwci_node_3] -> combine wci dwci/8(dwci_node_3)
  Add18/1 -> Mux159/2
  Integrator14/1 -> Display137/1, Demux99/1, [d_ui_hat_node_5]
  trans to column100/1(y) -> [V_Phi_Rei_squ_p_min_1_node_5], Display153/1
  [ui_tilt_node_5] -> Abs24/1
  [dwci_node_5] -> combine wci dwci/10(dwci_node_5)
  Constant364/1 -> Mux159/3
  Constant560/1 -> Mux170/3
  [ui_n_1] -> Demux118/1
  Integrator11/1 -> Display134/1, Demux98/1, [d_ui_hat_node_4]
  Interpreted MATLAB Function82/1 -> trans to column85/1(x)
  Integrator3/1 -> Demux130/1, Display125/1, [d_ui_hat_node_1]
  [ui_squ_5_node_5] -> cal sig25/1(x)
  Mux149/1 -> Interpreted MATLAB Function69/1
  Add21/1 -> Mux164/2
  [wei_vec] -> cal S_bar agent 4/4(wei_vec)
  [Qei_vec] -> Qei dynam agent 2/1(Qei_vec)
  Add22/1 -> Mux137/2
  Constant419/1 -> Mux204/3
  Constant363/1 -> Mux162/3
  [wei_3] -> Integrator19/1
  Constant596/1 -> cal d_theta_hat/1(c1)
  Constant398/1 -> cal Phi_bar_psi_e agent 2/4(thr_p_plus_1)
  Constant380/1 -> Add20/2
  trans to column88/1(y) -> [ui_squ_6_node_5]
  Interpreted MATLAB Function111/1 -> trans to column113/1(x)
  [ui_tilt_node_5] -> cal sig24/2(y)
  Mux159/1 -> Interpreted MATLAB Function88/1
  Demux99/1 -> d_ui_hat_node_5/1
  cal sig27/1(z) -> [ui_sig_2_node_5]
  Constant526/1 -> cal taui agent 1/5(Ji)
  [Phi_psi_e_node_3] -> combine Phi_psi_e/3(Phi_psi_e_node_3)
  [ui_sig_5_node_3] -> cal d_theta_hat2/9(ui_sig_5)
  Demux105/2 -> wci_node_1/2
  Interpreted MATLAB Function80/1 -> trans to column80/1(x)
  trans to column85/1(y) -> [ui_squ_1_node_5]
  cal Rei agent 3/1(Rei_3) -> [Rei_3]
  [ui_sig_5_node_5] -> cal d_theta_hat4/9(ui_sig_5)
  Abs28/1 -> Mux163/1
  cal d_sigma_w agent 2/1(d_sigma_w_2) -> Integrator47/1
  trans to column67/1(y) -> [ui_squ_4_node_2]
  [ui_squ_4_node_5] -> cal sig24/1(x)
  Interpreted MATLAB Function102/1 -> trans to column103/1(x)
  Constant521/1 -> Mux147/2
  Integrator15/1 -> Display138/1, Demux104/1, [d2_ui_hat_node_5]
  Constant324/1 -> Mux154/3
  cal sig17/1(z) -> [ui_sig_6_node_3]
  Interpreted MATLAB Function/1 -> trans to column116/1(x)
  Constant406/1 -> Mux206/3
  trans to column82/1(y) -> [ui_squ_5_node_5]
  [Qci_2] -> combine Qci Rci/2(Qci_2)
  [ui_squ_4_node_1] -> cal sig4/1(x)
  [ui_squ_5_node_4] -> cal sig19/1(x)
  [d2uihat_vec] -> cal wci dwci agent 2/3(d2uihat_vec)
  cal sig6/1(z) -> [ui_sig_1_node_2]
  combine tau/1(taui_vec) -> [taui_vec]
  [ui_sig_1_node_4] -> cal d_theta_hat3/5(ui_sig_1)
  [Qi_vec] -> Qi dynam agent 2/1(Qi_vec)
  [V_Phi_Rei_squ_p_min_1_node_5] -> combine V_Phi_Rei_squ_p_min_1/5(V_Phi_Rei_squ_p_min_1_node_5)
  [Si_squ_beta_w_2_vec] -> cal theta_Si_beta_w agent 5/3(Si_squ_beta_w_2_vec)
  [d_ui_hat_node_4] -> cal d_theta_hat3/11(dui_hat)
  cal dw_hat agent 5/1(dw_hat_5) -> [dw_hat_5]
  Demux125/2 -> Mux182/2
  [ui_hat_node_5] -> Add19/1
  [sigma_bar_w_hat_vec] -> cal dw_hat agent 3/4(sigma_bar_w_hat_vec)
  Constant360/1 -> Product8/1
  Mux172/1 -> Scope2/2
  Constant316/1 -> Product7/1
  [d_ui_hat_node_3] -> cal d_theta_hat2/11(dui_hat)
  Constant306/1 -> Add28/1
  [ui_sig_6_node_4] -> cal d_theta_hat3/10(ui_sig_6)
  cal Rei agent 2/1(Rei_2) -> [Rei_2]
  Integrator10/1 -> [ui_hat_node_4], Display133/1
  cal abs 87/1(y) -> Mux210/1
  [ui_sig_3_node_2] -> cal d_theta_hat1/7(ui_sig_3)
  Demux122/3 -> Mux175/1
  [V_Phi_Rei_div_pi_vec] -> choose ksi_est_err 41/1(x)
  [wi_4] -> combine dwi/4(wi_4)
  [ui_tilt_node_4] -> Abs20/1
  Interpreted MATLAB Function99/1 -> trans to column100/1(x)
  Interpreted MATLAB Function87/1 -> trans to column87/1(x)
  [wei_vec] -> cal Fi_S agent 1/5(wei_vec)
  Product6/1 -> Add17/2
  Add19/1 -> Demux128/1, [ui_tilt_node_5]
  [Qei_vec] -> cal Rei agent 2/1(Qei_vec)
  [sigma_bar_w_vec] -> cal d_sigma_w agent 3/5(sigma_w_bar_vec)
  cal dw_hat agent 3/1(dw_hat_3) -> [dw_hat_3]
  Constant579/1 -> cal Phi_psi_e agent 2/1(beta_Phi_1)
  cal differentiator d_sigma_bar_w_hat agent 1/1(Out1) -> Display164/1, [sigma_bar_w_est_1]
  Constant329/1 -> Product6/1
  Constant365/1 -> Add18/1
  trans to column81/1(y) -> [ui_squ_6_node_4]
  [ui_tilt_node_5] -> cal sig28/2(y)
  cal d_theta_hat1/1(d_ui_hat) -> Integrator1/1
  cal sig20/1(z) -> [ui_sig_1_node_4]
  Constant347/1 -> Product9/1
  [wei_vec] -> Qei dynam agent 5/2(wei_vec)
  [ui_squ_5_node_2] -> cal sig11/1(x)
  wi dynam agent 3/1(dwi_3) -> Integrator23/1
  Abs22/1 -> Mux156/1
  [wei_vec] -> cal Phi_bar_psi_e agent 5/7(wei_vec)
  [ui_tilt_node_5] -> cal sig29/2(y)
  Add10/1 -> Mux191/2
  cal differentiator d_sigma_bar_w_hat agent 2/3(Out3) -> Demux133/1, [d2_sigma_bar_w_est_2], Display113/1
  Abs18/1 -> Mux152/1
  cal sig24/1(z) -> [ui_sig_4_node_5]
  choose ksi_est_err 54/1(y) -> cal abs 74/1(x)
  trans to column122/1(y) -> [Si_squ_beta_w_1_node_5], Display163/1
  Abs21/1 -> Mux154/1
  Constant416/1 -> Mux208/3
  Constant345/1 -> Mux152/3
  cal Phi_bar_psi_e agent 2/1(Phi_bar_psi_e_node_2) -> [Phi_bar_psi_e_node_2]
  trans to column77/1(y) -> [ui_squ_2_node_4]
  Mux157/1 -> Interpreted MATLAB Function80/1
  cal sig21/1(z) -> [ui_sig_2_node_4]
  Constant574/1 -> cal Phi_psi_e agent 1/2(beta_Phi_2)
  [Rci_5] -> combine Qci Rci/10(Rci_5)
  cal theta_sigma_bar_w_tilt agent 2/2(theta_sigma_bar_w_tilt_2_2) -> [theta_sigma_bar_w_tilt_2_2]
  [d_sigma_bar_w_vec] -> cal sigma_bar_w_hat agent 3/5(d_sigma_bar_w_vec)
  trans to column76/1(y) -> [ui_squ_5_node_4]
  [V_Phi_Rei_div_pi_vec] -> choose ksi_est_err 74/1(x)
  Interpreted MATLAB Function77/1 -> trans to column76/1(x)
  [ui_tilt_node_4] -> cal sig23/2(y)
  Abs23/1 -> Mux157/1
  cal Ri agent 5/1(Ri_5) -> [Ri_5]
  [Si_squ_beta_w_1_node_4] -> combine Si_squ_beta_w_1/4(Si_squ_beta_w_1_node_4)
  Constant420/1 -> Mux203/2
  Interpreted MATLAB Function76/1 -> trans to column78/1(x)
  Demux129/1 -> d_ui_hat_node_3/1
  [wi_vec] -> cal d_sigma_w agent 5/3(wi_vec)
  Constant495/1 -> Mux194/3
  [dw_5] -> combine tau1/5(dw_5)
  Interpreted MATLAB Function79/1 -> trans to column79/1(x)
  cal sig4/1(z) -> [ui_sig_4_node_1]
  Demux116/2 -> wci_node_5/2
  Add13/1 -> Demux111/1, [ui_tilt_node_3]
  Demux124/3 -> Mux179/1
  [Fi_S_vec] -> cal taui agent 5/8(Fi_S_vec)
  Constant617/1 -> Product/1
  [V_Phi_Rei_div_pi_vec] -> choose ksi_est_err 71/1(x)
  [Qci_5] -> cal Rci agent 5/1(Qci_vec)
  Constant564/1 -> generate angular rate disturbance agent 3/1(dw_aa_t)
  Constant326/1 -> Mux156/2
  Mux153/1 -> Interpreted MATLAB Function77/1
  Mux175/1 -> Scope13/3
  Demux127/1 -> Mux184/2
  Constant435/1 -> cal sigma_bar_w_hat agent 2/1(h1w)
  [ui_tilt_node_4] -> cal sig21/2(y)
  Constant611/1 -> cal Si agent 2/1(cS0)
  [ui_tilt_node_4] -> Abs19/1
  trans to column124/1(y) -> [ui_squ_4_node_1]
  trans to column91/1(y) -> [V_Phi_Rei_squ_p_plus_1_node_4], Display120/1
  [ui_tilt_node_4] -> cal sig19/2(y)
  [wi_vec] -> wi dynam agent 3/2(wi_vec)
  [wi_vec] -> cal Fi_S agent 3/3(wi_vec)
  cal Rei agent 5/1(Rei_5) -> [Rei_5]
  cal Rci agent 4/1(Rci_4) -> [Rci_4]
  [ui_tilt_node_3] -> Abs15/1
  Interpreted MATLAB Function74/1 -> trans to column74/1(x)
  Constant626/1 -> Mux140/2
  [ui_tilt_node_3] -> cal sig13/2(y)
  [taui_vec] -> wi dynam agent 1/3(taui_vec)
  Constant590/1 -> Mux202/3
  [wi_vec] -> cal d_sigma_w agent 4/3(wi_vec)
  Constant301/1 -> Product5/1
  Constant314/1 -> Product4/1
  Constant308/1 -> Mux148/3
  Mux139/1 -> Interpreted MATLAB Function68/1
  combine Qci Rci1/1(V_Phi_Rei_vec) -> Memory12/1
  Constant633/1 -> Mux143/3
  Constant373/1 -> Add28/2
  [ui_tilt_node_2] -> cal sig11/2(y)
  Qei dynam agent 5/1(dQei_5) -> Integrator35/1
  Interpreted MATLAB Function123/1 -> trans to column124/1(x)
  Mux212/1 -> Interpreted MATLAB Function120/1
  cal wei agent 3/1(wei_3) -> [wei_3]
  [V_Phi_Rei_squ_p_plus_1_vec] -> cal Phi_bar_psi_e agent 5/11(V_Phi_Rei_squ_p_plus_1_vec)
  [duihat_vec] -> cal wci dwci agent 3/2(duihat_vec)
  cal abs 75/1(y) -> Mux188/1
  cal abs 62/1(y) -> Mux168/1
  [wei_5] -> Integrator44/1
  choose ksi_est_err 58/1(y) -> cal abs 78/1(x)
  cal Ri agent 1/1(Ri_1) -> [Ri_1]
  [theta_Si_beta_w_2_vec] -> cal taui agent 4/10(theta_Si_beta_w_2_vec)
  [Phi_psi_e_node_1] -> combine Phi_psi_e/1(Phi_psi_e_node_1)
  [Si_squ_beta_w_1_vec] -> cal theta_Si_beta_w agent 1/2(Si_squ_beta_w_1_vec)
  [Phi_psi_e_node_2] -> combine Phi_psi_e/2(Phi_psi_e_node_2)
  [ui_vec] -> cal wci dwci agent 3/1(ui_vec)
  [wei_4] -> combine wei Qei Rei/4(wei_4)
  Interpreted MATLAB Function93/1 -> trans to column93/1(x)
  Constant440/1 -> cal sigma_bar_w_hat agent 4/1(h1w)
  [dwci_node_4] -> combine wci dwci/9(dwci_node_4)
  Demux113/3 -> dwci_node_3/3
  Memory3/1 -> [Qi_vec]
  [duihat_vec] -> cal wci dwci agent 2/2(duihat_vec)
  [ui_squ_3_node_2] -> cal sig8/1(x)
  cal wci dwci agent 2/1(wci) -> Demux107/1, Display144/1, [wci_node_2]
  Constant641/1 -> Mux145/3
  Mux207/1 -> Interpreted MATLAB Function113/1
  cal theta_Si_beta_w agent 3/2(theta_Si_beta_w_2_node_3) -> [theta_Si_beta_w_2_node_3]
  combine S_bar/1(S_bar_vec) -> Memory11/1
  Abs14/1 -> Mux149/1
  Demux101/1 -> d2_ui_hat_node_2/1
  Constant359/1 -> Add21/1
  Demux115/3 -> dwci_node_4/3
  [ui_hat_node_2] -> Demux119/1
  [tsim] -> generate angular rate disturbance agent 4/4(t)
  Interpreted MATLAB Function98/1 -> trans to column99/1(x)
  [S_bar_node_5] -> combine S_bar/5(S_bar_node_5)
  Constant317/1 -> Mux153/3
  cal wci dwci agent 2/2(dwci) -> Display145/1, Demux109/1, [dwci_node_2]
  Demux107/2 -> wci_node_2/2
  [ui_tilt_node_5] -> cal sig25/2(y)
  [V_Phi_Rei_squ_p_plus_1_vec] -> cal Phi_bar_psi_e agent 2/11(V_Phi_Rei_squ_p_plus_1_vec)
  Demux127/2 -> Mux185/2
  trans to column71/1(y) -> [ui_squ_1_node_3]
  cal sig16/1(z) -> [ui_sig_3_node_3]
  Constant563/1 -> generate angular rate disturbance agent 2/3(dw_phi_t)
  Demux120/3 -> ui_tilt_node_4/3
  cal Fi_S agent 5/1(Fi_S_5) -> [Fi_S_5]
  [V_Phi_Rei_squ_p_plus_1_node_2] -> combine V_Phi_Rei_squ_p_plus_1/2(V_Phi_Rei_squ_p_plus_1_node_2)
  choose ksi_est_err 70/1(y) -> cal abs 90/1(x)
  Abs7/1 -> Mux141/1
  cal combine sigma_bar_w_tilt/1(sigma_bar_w_tilt_vec) -> [sigma_bar_w_tilt_vec]
  choose ksi_est_err 41/1(y) -> cal abs 61/1(x)
  [ui_vec] -> cal wci dwci agent 1/1(ui_vec)
  Memory8/1 -> [Rei_vec]
  [d2_ui_hat_node_1] -> combine duihat d2uihat/6(d2_ui_hat_node_1)
  Constant627/1 -> cal d_theta_hat1/1(c1)
  combine duihat d2uihat/2(d2uihat_vec) -> [d2uihat_vec]
  combine duihat d2uihat/1(duihat_vec) -> [duihat_vec]
  Constant559/1 -> generate angular rate disturbance agent 1/3(dw_phi_t)
  Constant453/1 -> cal dw_hat agent 4/1(h3w)
  Product2/1 -> Add25/2
  [d_ui_hat_node_5] -> combine duihat d2uihat/5(d_ui_hat_node_5)
  Abs8/1 -> Mux143/1
  trans to column119/1(y) -> [Si_squ_beta_w_2_node_4], Display160/1
  Constant388/1 -> cal S_bar agent 3/2(gamma0)
  cal d_theta_hat4/3(d_d2ui_hat) -> Integrator15/1
  cal theta_sigma_bar_w_tilt agent 3/2(theta_sigma_bar_w_tilt_2_3) -> [theta_sigma_bar_w_tilt_2_3]
  [ui_tilt_node_2] -> Abs9/1
  Constant517/1 -> Mux214/3
  [Ri_1] -> combine Qi Ri/6(Ri_1)
  [Phi_psi_e_vec] -> cal Si agent 2/3(Phi_psi_e_vec)
  [tau_1] -> combine tau/1(tau_1)
  [V_Phi_Rei_div_pi_vec] -> cal Phi_psi_e agent 4/7(V_Phi_Rei_div_pi_vec)
  cal sig7/1(z) -> [ui_sig_2_node_2]
  [dw_2] -> combine tau1/2(dw_2)
  [Rei_4] -> combine wei Qei Rei/14(Rei_4)
  Constant512/1 -> Mux211/3
  [ui_squ_2_node_2] -> cal sig7/1(x)
  [Rci_vec] -> cal wci dwci agent 3/4(Rci_mat)
  [ui_squ_1_node_1] -> cal sig/1(x)
  cal wci dwci agent 1/2(dwci) -> Display143/1, Demux106/1, [dwci_node_1]
  Demux121/2 -> Mux186/2
  [ui_vec] -> choose ui agent 1/1(x)
  cal d_theta_hat4/1(d_ui_hat) -> Integrator13/1
  Abs10/1 -> Mux139/1
  [dw_hat_vec] -> cal error dw_tilt/2(dw_hat_vec)
  Integrator2/1 -> Display124/1, [ui_hat_node_1]
  [Qei_vec] -> Qei dynam agent 1/1(Qei_vec)
  cal Rei agent 1/1(Rei_1) -> [Rei_1]
  cal abs 95/1(y) -> Mux170/1
  [d2_ui_hat_node_2] -> combine duihat d2uihat/7(d2_ui_hat_node_2)
  Constant612/1 -> cal Si agent 3/1(cS0)
  [ui_sig_5_node_1] -> cal d_theta_hat/9(ui_sig_5)
  cal differentiator d_sigma_bar_w_hat agent 3/3(Out3) -> Demux135/1, [d2_sigma_bar_w_est_3], Display116/1
  trans to column116/1(y) -> [ui_squ_1_node_1]
  Constant395/1 -> cal Phi_bar_psi_e agent 2/1(pp0)
  Constant601/1 -> Mux191/3
  [sigma_bar_w_tilt_vec] -> choose ksi_est_err 53/1(x)
  Abs1/1 -> Mux191/1
  [Si_2] -> combine Si/2(Si_2)
  trans to column84/1(y) -> [ui_squ_2_node_5]
  [ui_tilt_node_1] -> Abs3/1
  Constant616/1 -> Add11/1
  Abs4/1 -> Mux137/1
  cal abs 63/1(y) -> Mux199/1
  [ui_tilt_node_1] -> cal sig4/2(y)
  Constant391/1 -> cal Phi_bar_psi_e agent 1/3(beta_Phi_2)
  Qi dynam agent 3/1(dQi_3) -> Integrator28/1
  Constant355/1 -> Mux165/2
  [ui_squ_1_node_2] -> cal sig6/1(x)
  [sigma_bar_w_tilt_squ_2_3] -> cal theta_sigma_bar_w_tilt agent 3/3(sigma_bar_w_tilt_squ_2_3)
  Product/1 -> Add11/2
  [wi_vec] -> cal wei agent 2/1(wi_vec)
  [d_ui_hat_node_4] -> combine duihat d2uihat/4(d_ui_hat_node_4)
  trans to column66/1(y) -> [ui_squ_3_node_2]
  combine Si_squ_beta_w_1/1(Si_squ_beta_w_1_vec) -> Memory21/1
  [sigma_bar_w_vec] -> cal d_sigma_w agent 1/5(sigma_w_bar_vec)
  [V_Phi_Rei_squ_2p_vec] -> cal Phi_bar_psi_e agent 2/12(V_Phi_Rei_squ_2p_vec)
  [ui_tilt_node_1] -> Abs1/1
  Abs2/1 -> Mux213/1
  [ui_tilt_node_4] -> cal sig22/2(y)
  Constant591/1 -> Mux137/3
  [theta_sigma_bar_w_tilt_1_vec] -> cal sigma_bar_w_hat agent 5/3(theta_sigma_bar_w_tilt_1_vec)
  [V_Phi_Rei_squ_p_plus_1_vec] -> cal S_bar agent 5/6(V_Phi_Rei_squ_p_plus_1_vec)
  Demux130/2 -> d_ui_hat_node_1/2
  [sigma_bar_w_tilt_squ_2_1] -> cal theta_sigma_bar_w_tilt agent 1/3(sigma_bar_w_tilt_squ_2_1)
  Constant622/1 -> Mux139/3
  Mux202/1 -> Interpreted MATLAB Function/1
  Constant618/1 -> cal d_theta_hat/4(chi_t)
  [sigma_bar_w_vec] -> cal differentiator d_sigma_bar_w_hat agent 2/1(x)
  [Rci_2] -> combine Qci Rci/7(Rci_2)
  [V_Phi_Rei_squ_p_min_1_vec] -> cal Phi_bar_psi_e agent 3/10(V_Phi_Rei_squ_p_min_1_vec)
  [Rei_vec] -> cal wei agent 5/2(Rei_vec)
  Constant595/1 -> Mux138/2
  [ui_tilt_node_4] -> Abs21/1
  [dw_hat_vec] -> cal taui agent 3/7(dw_hat_vec)
  [ui_sig_5_node_2] -> cal d_theta_hat1/9(ui_sig_5)
  Constant593/1 -> Product1/1
  Qi dynam agent 2/1(dQi_2) -> Integrator27/1
  Constant514/1 -> Mux210/3
  cal Phi_psi_e agent 5/1(Phi_psi_e_node_5) -> [Phi_psi_e_node_5]
  [ui_sig_1_node_1] -> cal d_theta_hat/5(ui_sig_1)
  Constant397/1 -> cal Phi_bar_psi_e agent 2/3(beta_Phi_2)
  [ui_tilt_node_5] -> Abs25/1
  [ui_sig_4_node_3] -> cal d_theta_hat2/8(ui_sig_4)
  choose ksi_est_err 62/1(y) -> cal abs 82/1(x)
  combine Si_squ_beta_w_2/1(Si_squ_beta_w_2_vec) -> Memory22/1
  Mux144/1 -> Interpreted MATLAB Function67/1
  [wei_vec] -> Qei dynam agent 2/2(wei_vec)
  [wei_vec] -> cal Si agent 1/2(wei_vec)
  Mux138/1 -> Interpreted MATLAB Function62/1
  cal differentiator d_sigma_bar_w_hat agent 1/3(Out3) -> Demux131/1, [d2_sigma_bar_w_est_1], Display108/1
  [Rei_5] -> combine wei Qei Rei/15(Rei_5)
  Demux103/1 -> d2_ui_hat_node_4/1
  Memory21/1 -> [Si_squ_beta_w_1_vec]
  [d2_ui_hat_node_4] -> combine duihat d2uihat/9(d2_ui_hat_node_4)
  trans to column69/1(y) -> [ui_squ_5_node_3]
  [ui_sig_4_node_1] -> cal d_theta_hat/8(ui_sig_4)
  [Phi_bar_psi_e_vec] -> cal Fi_S agent 5/8(Phi_bar_psi_e_vec)
  [V_Phi_Rei_3] -> combine Qci Rci1/3(V_Phi_Rei_3)
  Abs/1 -> Mux202/1
  Abs26/1 -> Mux162/1
  Constant403/1 -> cal theta_sigma_bar_w_tilt agent 1/1(alfa_theta_obs_w)
  Demux115/1 -> dwci_node_4/1
  cal wci dwci agent 3/1(wci) -> Display146/1, Demux112/1, [wci_node_3]
  Interpreted MATLAB Function122/1 -> trans to column123/1(x)
  [ui_tilt_node_1] -> Abs2/1
  Constant557/1 -> generate angular rate disturbance agent 1/1(dw_aa_t)
  Constant405/1 -> cal theta_sigma_bar_w_tilt agent 2/1(alfa_theta_obs_w)
  [ui_squ_2_node_3] -> cal sig15/1(x)
  Mux171/1 -> Scope2/1
  Constant594/1 -> Mux138/3
  Constant625/1 -> Mux140/3
  cal sig3/1(z) -> [ui_sig_6_node_1]
  [d_ui_hat_node_1] -> combine duihat d2uihat/1(d_ui_hat_node_1)
  [V_Phi_Rei_squ_p_plus_1_vec] -> cal S_bar agent 3/6(V_Phi_Rei_squ_p_plus_1_vec)
  Demux104/2 -> d2_ui_hat_node_5/2
  Abs20/1 -> Mux155/1
  Constant386/1 -> wi dynam agent 4/1(Ji)
  Mux209/1 -> Interpreted MATLAB Function117/1
  Constant540/1 -> cal taui agent 5/1(c_w_1)
  [V_Phi_Rei_squ_2p_vec] -> cal Phi_bar_psi_e agent 5/12(V_Phi_Rei_squ_2p_vec)
  [sigma_w_1] -> combine sigma_w/1(sigma_w_1)
  cal Qci agent 4/1(Qci_4) -> [Qci_4]
  [S_bar_vec] -> cal Phi_bar_psi_e agent 5/8(S_bar_vec)
  [ui_sig_6_node_1] -> cal d_theta_hat/10(ui_sig_6)
  Add29/1 -> Mux151/2
  Integrator13/1 -> Display136/1, [ui_hat_node_5]
  Demux106/2 -> dwci_node_1/2
  trans to column105/1(y) -> [ui_squ_2_node_1]
  [ui_sig_2_node_1] -> cal d_theta_hat/6(ui_sig_2)
  cal sig/1(z) -> [ui_sig_1_node_1]
  Product1/1 -> Add22/2
  [wei_2] -> Integrator17/1
  [ui_squ_6_node_1] -> cal sig3/1(x)
  Constant370/1 -> Product1/2
  trans to column94/1(y) -> [V_Phi_Rei_squ_2p_node_2], Display99/1
  Interpreted MATLAB Function110/1 -> trans to column112/1(x)
  Constant609/1 -> cal Si agent 1/1(cS0)
  Constant358/1 -> Mux164/3
  combine theta_sigma_bar_w_tilt/2(theta_sigma_bar_w_tilt_2_vec) -> [theta_sigma_bar_w_tilt_2_vec]
  Abs13/1 -> Mux146/1
  Interpreted MATLAB Function62/1 -> trans to column62/1(x)
  Constant511/1 -> Mux211/2
  Constant603/1 -> Mux213/2
  choose ksi_est_err 71/1(y) -> cal abs 91/1(x)
  Qi dynam agent 4/1(dQi_4) -> Integrator29/1
  [V_Phi_Rei_squ_p_min_1_node_1] -> combine V_Phi_Rei_squ_p_min_1/1(V_Phi_Rei_squ_p_min_1_node_1)
  [duihat_vec] -> cal wci dwci agent 1/2(duihat_vec)
  Qei dynam agent 3/1(dQei_3) -> Integrator33/1
  [ui_tilt_node_1] -> cal sig/2(y)
  cal Ri agent 3/1(Ri_3) -> [Ri_3]
  Integrator12/1 -> Display135/1, Demux103/1, [d2_ui_hat_node_4]
  Constant410/1 -> Mux136/3
  [theta_Si_beta_w_1_vec] -> cal taui agent 5/9(theta_Si_beta_w_1_vec)
  Interpreted MATLAB Function70/1 -> trans to column69/1(x)
  Demux116/1 -> wci_node_5/1
  [V_Phi_Rei_squ_p_plus_1_vec] -> cal Phi_bar_psi_e agent 1/11(V_Phi_Rei_squ_p_plus_1_vec)
  combine wei Qei Rei/2(Qei_vec) -> Memory7/1
  [d_ui_hat_node_1] -> cal d_theta_hat/11(dui_hat)
  Demux132/2 -> d_sigma_bar_w_est_1/2
  Constant369/1 -> Product/2
  Demux104/1 -> d2_ui_hat_node_5/1
  control input generator agent 3/1(ui) -> [ui_n_3]
  control input generator agent 4/1(ui) -> [ui_n_4]
  [u0] -> control input generator agent 4/1(u0)
  [u0] -> control input generator agent 1/1(u0)
  control input generator agent 5/1(ui) -> [ui_n_5]
  [u0] -> control input generator agent 5/1(u0)
  Memory/1 -> [ui_vec]
  combine norminal formation control input/1(ui_vec) -> Memory/1
  [ui_n_4] -> combine norminal formation control input/4(ui_4)
  [ui_n_2] -> combine norminal formation control input/2(ui_2)
  [ui_n_1] -> combine norminal formation control input/1(ui_1)
  [u0] -> control input generator agent 2/1(u0)
  control input generator agent 1/1(ui) -> [ui_n_1]
  [ui_n_5] -> combine norminal formation control input/5(ui_5)
  control input generator agent 2/1(ui) -> [ui_n_2]
  [ui_n_3] -> combine norminal formation control input/3(ui_3)
  [u0] -> control input generator agent 3/1(u0)
  [Phi_psi_e_vec] -> To Workspace31/1
  [Qci_vec] -> To Workspace26/1
  [Si_vec] -> To Workspace37/1
  [dw_tilt_vec] -> To Workspace25/1
  [wi_vec] -> To Workspace34/1
  [wci_vec] -> To Workspace23/1
  [sigma_bar_w_hat_vec] -> To Workspace27/1
  [wei_vec] -> To Workspace28/1
  [dw_hat_vec] -> To Workspace39/1
  [S_bar_vec] -> To Workspace36/1
  [sigma_w_vec] -> To Workspace29/1
  [Qi_vec] -> To Workspace35/1
  [dw_vec] -> To Workspace38/1
  [sigma_bar_w_vec] -> To Workspace30/1
  [V_Phi_Rei_vec] -> To Workspace24/1
  [Qei_vec] -> To Workspace33/1
  [Phi_bar_psi_e_vec] -> To Workspace32/1
  Constant64/1 -> leader control input/3(T2)
  [V_init_out] -> leader eta0 Integrator/3
  Constant130/1 -> process velocity/7(R1)
  Clock/1 -> [tsim]
  Constant132/1 -> process velocity/10(Rz2)
  Constant65/1 -> leader control input/4(R0)
  Demux1/1 -> ksi_0/1
  [u0] -> leader eta0 Integrator/1
  Constant/1 -> leader control input/2(T1)
  leader eta0 Integrator/1 -> [eta0], leader ksi0 Integrator/1
  [eta0] -> Demux22/1
  Demux1/2 -> ksi_0/2
  Demux22/2 -> eta_0/2
  [ksi0] -> Demux1/1
  [tsim] -> process velocity/11(t)
  Demux22/1 -> eta_0/1
  Constant133/1 -> process velocity/9(Ry2)
  leader control input/1(u0) -> [u0]
  Step/1 -> leader eta0 Integrator/2
  Constant73/1 -> process velocity/5(PZ1)
  Constant71/1 -> process velocity/2(T1)
  Constant131/1 -> process velocity/1(T0)
  Constant67/1 -> leader control input/6(Rx2)
  Constant72/1 -> process velocity/4(PZ0)
  Constant68/1 -> leader control input/7(Ry2)
  Constant129/1 -> process velocity/6(R0)
  Demux1/3 -> ksi_0/3
  Constant70/1 -> process velocity/3(T2)
  Constant66/1 -> leader control input/5(R1)
  Constant134/1 -> process velocity/8(Rx2)
  [tsim] -> leader control input/1(t)
  leader ksi0 Integrator/1 -> [ksi0]
  Demux22/3 -> eta_0/3
  process velocity/1(V_init_out) -> [V_init_out]
  Constant69/1 -> leader control input/8(Rz2)
